simulink model "model"  (R2016a)
(part 2 of 2)

      | %<Name>
  bus13 : powerlib/Measurements/Load Flow Bus  LConnTagsString=a  Phases=single  Connectors=on one side  ID=bus13  Vbase=132000  Vref=1  Vangle=0  VLF=1  VLFb=1  VLFc=1  angleLF=0  angleLFb=0  angleLFc=0
      settings: AttributesFormatString=|
      | %<ID>
      | %<Vbase>V
      | %<VLF>pu
      | %<angleLF>deg.
      | %<Name>
  bus130 : powerlib/Measurements/Load Flow Bus  LConnTagsString=a  Phases=single  Connectors=on one side  ID=bus130  Vbase=220000  Vref=1  Vangle=0  VLF=1  VLFb=1  VLFc=1  angleLF=0  angleLFb=0  angleLFc=0
      settings: AttributesFormatString=|
      | %<ID>
      | %<Vbase>V
      | %<VLF>pu
      | %<angleLF>deg.
      | %<Name>
  bus131 : powerlib/Measurements/Load Flow Bus  LConnTagsString=a  Phases=single  Connectors=on one side  ID=bus131  Vbase=220000  Vref=1  Vangle=0  VLF=1  VLFb=1  VLFc=1  angleLF=0  angleLFb=0  angleLFc=0
      settings: AttributesFormatString=|
      | %<ID>
      | %<Vbase>V
      | %<VLF>pu
      | %<angleLF>deg.
      | %<Name>
  bus132 : powerlib/Measurements/Load Flow Bus  LConnTagsString=a  Phases=single  Connectors=on one side  ID=bus132  Vbase=220000  Vref=1  Vangle=0  VLF=1  VLFb=1  VLFc=1  angleLF=0  angleLFb=0  angleLFc=0
      settings: AttributesFormatString=|
      | %<ID>
      | %<Vbase>V
      | %<VLF>pu
      | %<angleLF>deg.
      | %<Name>
  bus133 : powerlib/Measurements/Load Flow Bus  LConnTagsString=a  Phases=single  Connectors=on one side  ID=bus133  Vbase=220000  Vref=1  Vangle=0  VLF=1  VLFb=1  VLFc=1  angleLF=0  angleLFb=0  angleLFc=0
      settings: AttributesFormatString=|
      | %<ID>
      | %<Vbase>V
      | %<VLF>pu
      | %<angleLF>deg.
      | %<Name>
  bus134 : powerlib/Measurements/Load Flow Bus  LConnTagsString=a  Phases=single  Connectors=on one side  ID=bus134  Vbase=220000  Vref=1  Vangle=0  VLF=1  VLFb=1  VLFc=1  angleLF=0  angleLFb=0  angleLFc=0
      settings: AttributesFormatString=|
      | %<ID>
      | %<Vbase>V
      | %<VLF>pu
      | %<angleLF>deg.
      | %<Name>
  bus135 : powerlib/Measurements/Load Flow Bus  LConnTagsString=a  Phases=single  Connectors=on one side  ID=bus135  Vbase=220000  Vref=1  Vangle=0  VLF=1  VLFb=1  VLFc=1  angleLF=0  angleLFb=0  angleLFc=0
      settings: AttributesFormatString=|
      | %<ID>
      | %<Vbase>V
      | %<VLF>pu
      | %<angleLF>deg.
      | %<Name>
  bus136 : powerlib/Measurements/Load Flow Bus  LConnTagsString=a  Phases=single  Connectors=on one side  ID=bus136  Vbase=220000  Vref=1  Vangle=0  VLF=1  VLFb=1  VLFc=1  angleLF=0  angleLFb=0  angleLFc=0
      settings: AttributesFormatString=|
      | %<ID>
      | %<Vbase>V
      | %<VLF>pu
      | %<angleLF>deg.
      | %<Name>
  bus137 : powerlib/Measurements/Load Flow Bus  LConnTagsString=a  Phases=single  Connectors=on one side  ID=bus137  Vbase=220000  Vref=1  Vangle=0  VLF=1  VLFb=1  VLFc=1  angleLF=0  angleLFb=0  angleLFc=0
      settings: AttributesFormatString=|
      | %<ID>
      | %<Vbase>V
      | %<VLF>pu
      | %<angleLF>deg.
      | %<Name>
  bus138 : powerlib/Measurements/Load Flow Bus  LConnTagsString=a  Phases=single  Connectors=on one side  ID=bus138  Vbase=220000  Vref=1  Vangle=0  VLF=1  VLFb=1  VLFc=1  angleLF=0  angleLFb=0  angleLFc=0
      settings: AttributesFormatString=|
      | %<ID>
      | %<Vbase>V
      | %<VLF>pu
      | %<angleLF>deg.
      | %<Name>
  bus139 : powerlib/Measurements/Load Flow Bus  LConnTagsString=a  Phases=single  Connectors=on one side  ID=bus139  Vbase=220000  Vref=1  Vangle=0  VLF=1  VLFb=1  VLFc=1  angleLF=0  angleLFb=0  angleLFc=0
      settings: AttributesFormatString=|
      | %<ID>
      | %<Vbase>V
      | %<VLF>pu
      | %<angleLF>deg.
      | %<Name>
  bus14 : powerlib/Measurements/Load Flow Bus  LConnTagsString=a  Phases=single  Connectors=on one side  ID=bus14  Vbase=132000  Vref=1  Vangle=0  VLF=1  VLFb=1  VLFc=1  angleLF=0  angleLFb=0  angleLFc=0
      settings: AttributesFormatString=|
      | %<ID>
      | %<Vbase>V
      | %<VLF>pu
      | %<angleLF>deg.
      | %<Name>
  bus140 : powerlib/Measurements/Load Flow Bus  LConnTagsString=a  Phases=single  Connectors=on one side  ID=bus140  Vbase=220000  Vref=1  Vangle=0  VLF=1  VLFb=1  VLFc=1  angleLF=0  angleLFb=0  angleLFc=0
      settings: AttributesFormatString=|
      | %<ID>
      | %<Vbase>V
      | %<VLF>pu
      | %<angleLF>deg.
      | %<Name>
  bus141 : powerlib/Measurements/Load Flow Bus  LConnTagsString=a  Phases=single  Connectors=on one side  ID=bus141  Vbase=220000  Vref=1  Vangle=0  VLF=1  VLFb=1  VLFc=1  angleLF=0  angleLFb=0  angleLFc=0
      settings: AttributesFormatString=|
      | %<ID>
      | %<Vbase>V
      | %<VLF>pu
      | %<angleLF>deg.
      | %<Name>
  bus142 : powerlib/Measurements/Load Flow Bus  LConnTagsString=a  Phases=single  Connectors=on one side  ID=bus142  Vbase=220000  Vref=1  Vangle=0  VLF=1  VLFb=1  VLFc=1  angleLF=0  angleLFb=0  angleLFc=0
      settings: AttributesFormatString=|
      | %<ID>
      | %<Vbase>V
      | %<VLF>pu
      | %<angleLF>deg.
      | %<Name>
  bus143 : powerlib/Measurements/Load Flow Bus  LConnTagsString=a  Phases=single  Connectors=on one side  ID=bus143  Vbase=220000  Vref=1  Vangle=0  VLF=1  VLFb=1  VLFc=1  angleLF=0  angleLFb=0  angleLFc=0
      settings: AttributesFormatString=|
      | %<ID>
      | %<Vbase>V
      | %<VLF>pu
      | %<angleLF>deg.
      | %<Name>
  bus144 : powerlib/Measurements/Load Flow Bus  LConnTagsString=a  Phases=single  Connectors=on one side  ID=bus144  Vbase=220000  Vref=1  Vangle=0  VLF=1  VLFb=1  VLFc=1  angleLF=0  angleLFb=0  angleLFc=0
      settings: AttributesFormatString=|
      | %<ID>
      | %<Vbase>V
      | %<VLF>pu
      | %<angleLF>deg.
      | %<Name>
  bus145 : powerlib/Measurements/Load Flow Bus  LConnTagsString=a  Phases=single  Connectors=on one side  ID=bus145  Vbase=220000  Vref=1  Vangle=0  VLF=1  VLFb=1  VLFc=1  angleLF=0  angleLFb=0  angleLFc=0
      settings: AttributesFormatString=|
      | %<ID>
      | %<Vbase>V
      | %<VLF>pu
      | %<angleLF>deg.
      | %<Name>
  bus146 : powerlib/Measurements/Load Flow Bus  LConnTagsString=a  Phases=single  Connectors=on one side  ID=bus146  Vbase=220000  Vref=1  Vangle=0  VLF=1  VLFb=1  VLFc=1  angleLF=0  angleLFb=0  angleLFc=0
      settings: AttributesFormatString=|
      | %<ID>
      | %<Vbase>V
      | %<VLF>pu
      | %<angleLF>deg.
      | %<Name>
  bus147 : powerlib/Measurements/Load Flow Bus  LConnTagsString=a  Phases=single  Connectors=on one side  ID=bus147  Vbase=220000  Vref=1  Vangle=0  VLF=1  VLFb=1  VLFc=1  angleLF=0  angleLFb=0  angleLFc=0
      settings: AttributesFormatString=|
      | %<ID>
      | %<Vbase>V
      | %<VLF>pu
      | %<angleLF>deg.
      | %<Name>
  bus148 : powerlib/Measurements/Load Flow Bus  LConnTagsString=a  Phases=single  Connectors=on one side  ID=bus148  Vbase=220000  Vref=1  Vangle=0  VLF=1  VLFb=1  VLFc=1  angleLF=0  angleLFb=0  angleLFc=0
      settings: AttributesFormatString=|
      | %<ID>
      | %<Vbase>V
      | %<VLF>pu
      | %<angleLF>deg.
      | %<Name>
  bus149 : powerlib/Measurements/Load Flow Bus  LConnTagsString=a  Phases=single  Connectors=on one side  ID=bus149  Vbase=220000  Vref=1  Vangle=0  VLF=1  VLFb=1  VLFc=1  angleLF=0  angleLFb=0  angleLFc=0
      settings: AttributesFormatString=|
      | %<ID>
      | %<Vbase>V
      | %<VLF>pu
      | %<angleLF>deg.
      | %<Name>
  bus15 : powerlib/Measurements/Load Flow Bus  LConnTagsString=a  Phases=single  Connectors=on one side  ID=bus15  Vbase=132000  Vref=1  Vangle=0  VLF=1  VLFb=1  VLFc=1  angleLF=0  angleLFb=0  angleLFc=0
      settings: AttributesFormatString=|
      | %<ID>
      | %<Vbase>V
      | %<VLF>pu
      | %<angleLF>deg.
      | %<Name>
  bus150 : powerlib/Measurements/Load Flow Bus  LConnTagsString=a  Phases=single  Connectors=on one side  ID=bus150  Vbase=220000  Vref=1  Vangle=0  VLF=1  VLFb=1  VLFc=1  angleLF=0  angleLFb=0  angleLFc=0
      settings: AttributesFormatString=|
      | %<ID>
      | %<Vbase>V
      | %<VLF>pu
      | %<angleLF>deg.
      | %<Name>
  bus151 : powerlib/Measurements/Load Flow Bus  LConnTagsString=a  Phases=single  Connectors=on one side  ID=bus151  Vbase=220000  Vref=1  Vangle=0  VLF=1  VLFb=1  VLFc=1  angleLF=0  angleLFb=0  angleLFc=0
      settings: AttributesFormatString=|
      | %<ID>
      | %<Vbase>V
      | %<VLF>pu
      | %<angleLF>deg.
      | %<Name>
  bus152 : powerlib/Measurements/Load Flow Bus  LConnTagsString=a  Phases=single  Connectors=on one side  ID=bus152  Vbase=220000  Vref=1  Vangle=0  VLF=1  VLFb=1  VLFc=1  angleLF=0  angleLFb=0  angleLFc=0
      settings: AttributesFormatString=|
      | %<ID>
      | %<Vbase>V
      | %<VLF>pu
      | %<angleLF>deg.
      | %<Name>
  bus153 : powerlib/Measurements/Load Flow Bus  LConnTagsString=a  Phases=single  Connectors=on one side  ID=bus153  Vbase=220000  Vref=1  Vangle=0  VLF=1  VLFb=1  VLFc=1  angleLF=0  angleLFb=0  angleLFc=0
      settings: AttributesFormatString=|
      | %<ID>
      | %<Vbase>V
      | %<VLF>pu
      | %<angleLF>deg.
      | %<Name>
  bus154 : powerlib/Measurements/Load Flow Bus  LConnTagsString=a  Phases=single  Connectors=on one side  ID=bus154  Vbase=220000  Vref=1  Vangle=0  VLF=1  VLFb=1  VLFc=1  angleLF=0  angleLFb=0  angleLFc=0
      settings: AttributesFormatString=|
      | %<ID>
      | %<Vbase>V
      | %<VLF>pu
      | %<angleLF>deg.
      | %<Name>
  bus155 : powerlib/Measurements/Load Flow Bus  LConnTagsString=a  Phases=single  Connectors=on one side  ID=bus155  Vbase=220000  Vref=1  Vangle=0  VLF=1  VLFb=1  VLFc=1  angleLF=0  angleLFb=0  angleLFc=0
      settings: AttributesFormatString=|
      | %<ID>
      | %<Vbase>V
      | %<VLF>pu
      | %<angleLF>deg.
      | %<Name>
  bus156 : powerlib/Measurements/Load Flow Bus  LConnTagsString=a  Phases=single  Connectors=on one side  ID=bus156  Vbase=220000  Vref=1  Vangle=0  VLF=1  VLFb=1  VLFc=1  angleLF=0  angleLFb=0  angleLFc=0
      settings: AttributesFormatString=|
      | %<ID>
      | %<Vbase>V
      | %<VLF>pu
      | %<angleLF>deg.
      | %<Name>
  bus157 : powerlib/Measurements/Load Flow Bus  LConnTagsString=a  Phases=single  Connectors=on one side  ID=bus157  Vbase=400000  Vref=1  Vangle=0  VLF=1  VLFb=1  VLFc=1  angleLF=0  angleLFb=0  angleLFc=0
      settings: AttributesFormatString=|
      | %<ID>
      | %<Vbase>V
      | %<VLF>pu
      | %<angleLF>deg.
      | %<Name>
  bus158 : powerlib/Measurements/Load Flow Bus  LConnTagsString=a  Phases=single  Connectors=on one side  ID=bus158  Vbase=400000  Vref=1  Vangle=0  VLF=1  VLFb=1  VLFc=1  angleLF=0  angleLFb=0  angleLFc=0
      settings: AttributesFormatString=|
      | %<ID>
      | %<Vbase>V
      | %<VLF>pu
      | %<angleLF>deg.
      | %<Name>
  bus159 : powerlib/Measurements/Load Flow Bus  LConnTagsString=a  Phases=single  Connectors=on one side  ID=bus159  Vbase=400000  Vref=1  Vangle=0  VLF=1  VLFb=1  VLFc=1  angleLF=0  angleLFb=0  angleLFc=0
      settings: AttributesFormatString=|
      | %<ID>
      | %<Vbase>V
      | %<VLF>pu
      | %<angleLF>deg.
      | %<Name>
  bus16 : powerlib/Measurements/Load Flow Bus  LConnTagsString=a  Phases=single  Connectors=on one side  ID=bus16  Vbase=132000  Vref=1  Vangle=0  VLF=1  VLFb=1  VLFc=1  angleLF=0  angleLFb=0  angleLFc=0
      settings: AttributesFormatString=|
      | %<ID>
      | %<Vbase>V
      | %<VLF>pu
      | %<angleLF>deg.
      | %<Name>
  bus160 : powerlib/Measurements/Load Flow Bus  LConnTagsString=a  Phases=single  Connectors=on one side  ID=bus160  Vbase=400000  Vref=1  Vangle=0  VLF=1  VLFb=1  VLFc=1  angleLF=0  angleLFb=0  angleLFc=0
      settings: AttributesFormatString=|
      | %<ID>
      | %<Vbase>V
      | %<VLF>pu
      | %<angleLF>deg.
      | %<Name>
  bus17 : powerlib/Measurements/Load Flow Bus  LConnTagsString=a  Phases=single  Connectors=on one side  ID=bus17  Vbase=132000  Vref=1  Vangle=0  VLF=1  VLFb=1  VLFc=1  angleLF=0  angleLFb=0  angleLFc=0
      settings: AttributesFormatString=|
      | %<ID>
      | %<Vbase>V
      | %<VLF>pu
      | %<angleLF>deg.
      | %<Name>
  bus18 : powerlib/Measurements/Load Flow Bus  LConnTagsString=a  Phases=single  Connectors=on one side  ID=bus18  Vbase=132000  Vref=1  Vangle=0  VLF=1  VLFb=1  VLFc=1  angleLF=0  angleLFb=0  angleLFc=0
      settings: AttributesFormatString=|
      | %<ID>
      | %<Vbase>V
      | %<VLF>pu
      | %<angleLF>deg.
      | %<Name>
  bus19 : powerlib/Measurements/Load Flow Bus  LConnTagsString=a  Phases=single  Connectors=on one side  ID=bus19  Vbase=132000  Vref=1  Vangle=0  VLF=1  VLFb=1  VLFc=1  angleLF=0  angleLFb=0  angleLFc=0
      settings: AttributesFormatString=|
      | %<ID>
      | %<Vbase>V
      | %<VLF>pu
      | %<angleLF>deg.
      | %<Name>
  bus2 : powerlib/Measurements/Load Flow Bus  LConnTagsString=a  Phases=single  Connectors=on one side  ID=bus2  Vbase=132000  Vref=1  Vangle=0  VLF=1  VLFb=1  VLFc=1  angleLF=0  angleLFb=0  angleLFc=0
      settings: AttributesFormatString=|
      | %<ID>
      | %<Vbase>V
      | %<VLF>pu
      | %<angleLF>deg.
      | %<Name>
  bus20 : powerlib/Measurements/Load Flow Bus  LConnTagsString=a  Phases=single  Connectors=on one side  ID=bus20  Vbase=132000  Vref=1  Vangle=0  VLF=1  VLFb=1  VLFc=1  angleLF=0  angleLFb=0  angleLFc=0
      settings: AttributesFormatString=|
      | %<ID>
      | %<Vbase>V
      | %<VLF>pu
      | %<angleLF>deg.
      | %<Name>
  bus21 : powerlib/Measurements/Load Flow Bus  LConnTagsString=a  Phases=single  Connectors=on one side  ID=bus21  Vbase=132000  Vref=1  Vangle=0  VLF=1  VLFb=1  VLFc=1  angleLF=0  angleLFb=0  angleLFc=0
      settings: AttributesFormatString=|
      | %<ID>
      | %<Vbase>V
      | %<VLF>pu
      | %<angleLF>deg.
      | %<Name>
  bus22 : powerlib/Measurements/Load Flow Bus  LConnTagsString=a  Phases=single  Connectors=on one side  ID=bus22  Vbase=132000  Vref=1  Vangle=0  VLF=1  VLFb=1  VLFc=1  angleLF=0  angleLFb=0  angleLFc=0
      settings: AttributesFormatString=|
      | %<ID>
      | %<Vbase>V
      | %<VLF>pu
      | %<angleLF>deg.
      | %<Name>
  bus23 : powerlib/Measurements/Load Flow Bus  LConnTagsString=a  Phases=single  Connectors=on one side  ID=bus23  Vbase=132000  Vref=1  Vangle=0  VLF=1  VLFb=1  VLFc=1  angleLF=0  angleLFb=0  angleLFc=0
      settings: AttributesFormatString=|
      | %<ID>
      | %<Vbase>V
      | %<VLF>pu
      | %<angleLF>deg.
      | %<Name>
  bus24 : powerlib/Measurements/Load Flow Bus  LConnTagsString=a  Phases=single  Connectors=on one side  ID=bus24  Vbase=132000  Vref=1  Vangle=0  VLF=1  VLFb=1  VLFc=1  angleLF=0  angleLFb=0  angleLFc=0
      settings: AttributesFormatString=|
      | %<ID>
      | %<Vbase>V
      | %<VLF>pu
      | %<angleLF>deg.
      | %<Name>
  bus25 : powerlib/Measurements/Load Flow Bus  LConnTagsString=a  Phases=single  Connectors=on one side  ID=bus25  Vbase=132000  Vref=1  Vangle=0  VLF=1  VLFb=1  VLFc=1  angleLF=0  angleLFb=0  angleLFc=0
      settings: AttributesFormatString=|
      | %<ID>
      | %<Vbase>V
      | %<VLF>pu
      | %<angleLF>deg.
      | %<Name>
  bus26 : powerlib/Measurements/Load Flow Bus  LConnTagsString=a  Phases=single  Connectors=on one side  ID=bus26  Vbase=220000  Vref=1  Vangle=0  VLF=1  VLFb=1  VLFc=1  angleLF=0  angleLFb=0  angleLFc=0
      settings: AttributesFormatString=|
      | %<ID>
      | %<Vbase>V
      | %<VLF>pu
      | %<angleLF>deg.
      | %<Name>
  bus27 : powerlib/Measurements/Load Flow Bus  LConnTagsString=a  Phases=single  Connectors=on one side  ID=bus27  Vbase=220000  Vref=1  Vangle=0  VLF=1  VLFb=1  VLFc=1  angleLF=0  angleLFb=0  angleLFc=0
      settings: AttributesFormatString=|
      | %<ID>
      | %<Vbase>V
      | %<VLF>pu
      | %<angleLF>deg.
      | %<Name>
  bus28 : powerlib/Measurements/Load Flow Bus  LConnTagsString=a  Phases=single  Connectors=on one side  ID=bus28  Vbase=220000  Vref=1  Vangle=0  VLF=1  VLFb=1  VLFc=1  angleLF=0  angleLFb=0  angleLFc=0
      settings: AttributesFormatString=|
      | %<ID>
      | %<Vbase>V
      | %<VLF>pu
      | %<angleLF>deg.
      | %<Name>
  bus29 : powerlib/Measurements/Load Flow Bus  LConnTagsString=a  Phases=single  Connectors=on one side  ID=bus29  Vbase=220000  Vref=1  Vangle=0  VLF=1  VLFb=1  VLFc=1  angleLF=0  angleLFb=0  angleLFc=0
      settings: AttributesFormatString=|
      | %<ID>
      | %<Vbase>V
      | %<VLF>pu
      | %<angleLF>deg.
      | %<Name>
  bus3 : powerlib/Measurements/Load Flow Bus  LConnTagsString=a  Phases=single  Connectors=on one side  ID=bus3  Vbase=132000  Vref=1  Vangle=0  VLF=1  VLFb=1  VLFc=1  angleLF=0  angleLFb=0  angleLFc=0
      settings: AttributesFormatString=|
      | %<ID>
      | %<Vbase>V
      | %<VLF>pu
      | %<angleLF>deg.
      | %<Name>
  bus30 : powerlib/Measurements/Load Flow Bus  LConnTagsString=a  Phases=single  Connectors=on one side  ID=bus30  Vbase=220000  Vref=1  Vangle=0  VLF=1  VLFb=1  VLFc=1  angleLF=0  angleLFb=0  angleLFc=0
      settings: AttributesFormatString=|
      | %<ID>
      | %<Vbase>V
      | %<VLF>pu
      | %<angleLF>deg.
      | %<Name>
  bus31 : powerlib/Measurements/Load Flow Bus  LConnTagsString=a  Phases=single  Connectors=on one side  ID=bus31  Vbase=220000  Vref=1  Vangle=0  VLF=1  VLFb=1  VLFc=1  angleLF=0  angleLFb=0  angleLFc=0
      settings: AttributesFormatString=|
      | %<ID>
      | %<Vbase>V
      | %<VLF>pu
      | %<angleLF>deg.
      | %<Name>
  bus32 : powerlib/Measurements/Load Flow Bus  LConnTagsString=a  Phases=single  Connectors=on one side  ID=bus32  Vbase=220000  Vref=1  Vangle=0  VLF=1  VLFb=1  VLFc=1  angleLF=0  angleLFb=0  angleLFc=0
      settings: AttributesFormatString=|
      | %<ID>
      | %<Vbase>V
      | %<VLF>pu
      | %<angleLF>deg.
      | %<Name>
  bus33 : powerlib/Measurements/Load Flow Bus  LConnTagsString=a  Phases=single  Connectors=on one side  ID=bus33  Vbase=220000  Vref=1  Vangle=0  VLF=1  VLFb=1  VLFc=1  angleLF=0  angleLFb=0  angleLFc=0
      settings: AttributesFormatString=|
      | %<ID>
      | %<Vbase>V
      | %<VLF>pu
      | %<angleLF>deg.
      | %<Name>
  bus34 : powerlib/Measurements/Load Flow Bus  LConnTagsString=a  Phases=single  Connectors=on one side  ID=bus34  Vbase=220000  Vref=1  Vangle=0  VLF=1  VLFb=1  VLFc=1  angleLF=0  angleLFb=0  angleLFc=0
      settings: AttributesFormatString=|
      | %<ID>
      | %<Vbase>V
      | %<VLF>pu
      | %<angleLF>deg.
      | %<Name>
  bus35 : powerlib/Measurements/Load Flow Bus  LConnTagsString=a  Phases=single  Connectors=on one side  ID=bus35  Vbase=220000  Vref=1  Vangle=0  VLF=1  VLFb=1  VLFc=1  angleLF=0  angleLFb=0  angleLFc=0
      settings: AttributesFormatString=|
      | %<ID>
      | %<Vbase>V
      | %<VLF>pu
      | %<angleLF>deg.
      | %<Name>
  bus36 : powerlib/Measurements/Load Flow Bus  LConnTagsString=a  Phases=single  Connectors=on one side  ID=bus36  Vbase=220000  Vref=1  Vangle=0  VLF=1  VLFb=1  VLFc=1  angleLF=0  angleLFb=0  angleLFc=0
      settings: AttributesFormatString=|
      | %<ID>
      | %<Vbase>V
      | %<VLF>pu
      | %<angleLF>deg.
      | %<Name>
  bus37 : powerlib/Measurements/Load Flow Bus  LConnTagsString=a  Phases=single  Connectors=on one side  ID=bus37  Vbase=220000  Vref=1  Vangle=0  VLF=1  VLFb=1  VLFc=1  angleLF=0  angleLFb=0  angleLFc=0
      settings: AttributesFormatString=|
      | %<ID>
      | %<Vbase>V
      | %<VLF>pu
      | %<angleLF>deg.
      | %<Name>
  bus38 : powerlib/Measurements/Load Flow Bus  LConnTagsString=a  Phases=single  Connectors=on one side  ID=bus38  Vbase=220000  Vref=1  Vangle=0  VLF=1  VLFb=1  VLFc=1  angleLF=0  angleLFb=0  angleLFc=0
      settings: AttributesFormatString=|
      | %<ID>
      | %<Vbase>V
      | %<VLF>pu
      | %<angleLF>deg.
      | %<Name>
  bus39 : powerlib/Measurements/Load Flow Bus  LConnTagsString=a  Phases=single  Connectors=on one side  ID=bus39  Vbase=220000  Vref=1  Vangle=0  VLF=1  VLFb=1  VLFc=1  angleLF=0  angleLFb=0  angleLFc=0
      settings: AttributesFormatString=|
      | %<ID>
      | %<Vbase>V
      | %<VLF>pu
      | %<angleLF>deg.
      | %<Name>
  bus4 : powerlib/Measurements/Load Flow Bus  LConnTagsString=a  Phases=single  Connectors=on one side  ID=bus4  Vbase=132000  Vref=1  Vangle=0  VLF=1  VLFb=1  VLFc=1  angleLF=0  angleLFb=0  angleLFc=0
      settings: AttributesFormatString=|
      | %<ID>
      | %<Vbase>V
      | %<VLF>pu
      | %<angleLF>deg.
      | %<Name>
  bus40 : powerlib/Measurements/Load Flow Bus  LConnTagsString=a  Phases=single  Connectors=on one side  ID=bus40  Vbase=220000  Vref=1  Vangle=0  VLF=1  VLFb=1  VLFc=1  angleLF=0  angleLFb=0  angleLFc=0
      settings: AttributesFormatString=|
      | %<ID>
      | %<Vbase>V
      | %<VLF>pu
      | %<angleLF>deg.
      | %<Name>
  bus41 : powerlib/Measurements/Load Flow Bus  LConnTagsString=a  Phases=single  Connectors=on one side  ID=bus41  Vbase=220000  Vref=1  Vangle=0  VLF=1  VLFb=1  VLFc=1  angleLF=0  angleLFb=0  angleLFc=0
      settings: AttributesFormatString=|
      | %<ID>
      | %<Vbase>V
      | %<VLF>pu
      | %<angleLF>deg.
      | %<Name>
  bus42 : powerlib/Measurements/Load Flow Bus  LConnTagsString=a  Phases=single  Connectors=on one side  ID=bus42  Vbase=220000  Vref=1  Vangle=0  VLF=1  VLFb=1  VLFc=1  angleLF=0  angleLFb=0  angleLFc=0
      settings: AttributesFormatString=|
      | %<ID>
      | %<Vbase>V
      | %<VLF>pu
      | %<angleLF>deg.
      | %<Name>
  bus43 : powerlib/Measurements/Load Flow Bus  LConnTagsString=a  Phases=single  Connectors=on one side  ID=bus43  Vbase=220000  Vref=1  Vangle=0  VLF=1  VLFb=1  VLFc=1  angleLF=0  angleLFb=0  angleLFc=0
      settings: AttributesFormatString=|
      | %<ID>
      | %<Vbase>V
      | %<VLF>pu
      | %<angleLF>deg.
      | %<Name>
  bus44 : powerlib/Measurements/Load Flow Bus  LConnTagsString=a  Phases=single  Connectors=on one side  ID=bus44  Vbase=220000  Vref=1  Vangle=0  VLF=1  VLFb=1  VLFc=1  angleLF=0  angleLFb=0  angleLFc=0
      settings: AttributesFormatString=|
      | %<ID>
      | %<Vbase>V
      | %<VLF>pu
      | %<angleLF>deg.
      | %<Name>
  bus45 : powerlib/Measurements/Load Flow Bus  LConnTagsString=a  Phases=single  Connectors=on one side  ID=bus45  Vbase=220000  Vref=1  Vangle=0  VLF=1  VLFb=1  VLFc=1  angleLF=0  angleLFb=0  angleLFc=0
      settings: AttributesFormatString=|
      | %<ID>
      | %<Vbase>V
      | %<VLF>pu
      | %<angleLF>deg.
      | %<Name>
  bus46 : powerlib/Measurements/Load Flow Bus  LConnTagsString=a  Phases=single  Connectors=on one side  ID=bus46  Vbase=220000  Vref=1  Vangle=0  VLF=1  VLFb=1  VLFc=1  angleLF=0  angleLFb=0  angleLFc=0
      settings: AttributesFormatString=|
      | %<ID>
      | %<Vbase>V
      | %<VLF>pu
      | %<angleLF>deg.
      | %<Name>
  bus47 : powerlib/Measurements/Load Flow Bus  LConnTagsString=a  Phases=single  Connectors=on one side  ID=bus47  Vbase=220000  Vref=1  Vangle=0  VLF=1  VLFb=1  VLFc=1  angleLF=0  angleLFb=0  angleLFc=0
      settings: AttributesFormatString=|
      | %<ID>
      | %<Vbase>V
      | %<VLF>pu
      | %<angleLF>deg.
      | %<Name>
  bus48 : powerlib/Measurements/Load Flow Bus  LConnTagsString=a  Phases=single  Connectors=on one side  ID=bus48  Vbase=220000  Vref=1  Vangle=0  VLF=1  VLFb=1  VLFc=1  angleLF=0  angleLFb=0  angleLFc=0
      settings: AttributesFormatString=|
      | %<ID>
      | %<Vbase>V
      | %<VLF>pu
      | %<angleLF>deg.
      | %<Name>
  bus49 : powerlib/Measurements/Load Flow Bus  LConnTagsString=a  Phases=single  Connectors=on one side  ID=bus49  Vbase=220000  Vref=1  Vangle=0  VLF=1  VLFb=1  VLFc=1  angleLF=0  angleLFb=0  angleLFc=0
      settings: AttributesFormatString=|
      | %<ID>
      | %<Vbase>V
      | %<VLF>pu
      | %<angleLF>deg.
      | %<Name>
  bus5 : powerlib/Measurements/Load Flow Bus  LConnTagsString=a  Phases=single  Connectors=on one side  ID=bus5  Vbase=132000  Vref=1  Vangle=0  VLF=1  VLFb=1  VLFc=1  angleLF=0  angleLFb=0  angleLFc=0
      settings: AttributesFormatString=|
      | %<ID>
      | %<Vbase>V
      | %<VLF>pu
      | %<angleLF>deg.
      | %<Name>
  bus50 : powerlib/Measurements/Load Flow Bus  LConnTagsString=a  Phases=single  Connectors=on one side  ID=bus50  Vbase=220000  Vref=1  Vangle=0  VLF=1  VLFb=1  VLFc=1  angleLF=0  angleLFb=0  angleLFc=0
      settings: AttributesFormatString=|
      | %<ID>
      | %<Vbase>V
      | %<VLF>pu
      | %<angleLF>deg.
      | %<Name>
  bus51 : powerlib/Measurements/Load Flow Bus  LConnTagsString=a  Phases=single  Connectors=on one side  ID=bus51  Vbase=220000  Vref=1  Vangle=0  VLF=1  VLFb=1  VLFc=1  angleLF=0  angleLFb=0  angleLFc=0
      settings: AttributesFormatString=|
      | %<ID>
      | %<Vbase>V
      | %<VLF>pu
      | %<angleLF>deg.
      | %<Name>
  bus52 : powerlib/Measurements/Load Flow Bus  LConnTagsString=a  Phases=single  Connectors=on one side  ID=bus52  Vbase=220000  Vref=1  Vangle=0  VLF=1  VLFb=1  VLFc=1  angleLF=0  angleLFb=0  angleLFc=0
      settings: AttributesFormatString=|
      | %<ID>
      | %<Vbase>V
      | %<VLF>pu
      | %<angleLF>deg.
      | %<Name>
  bus53 : powerlib/Measurements/Load Flow Bus  LConnTagsString=a  Phases=single  Connectors=on one side  ID=bus53  Vbase=220000  Vref=1  Vangle=0  VLF=1  VLFb=1  VLFc=1  angleLF=0  angleLFb=0  angleLFc=0
      settings: AttributesFormatString=|
      | %<ID>
      | %<Vbase>V
      | %<VLF>pu
      | %<angleLF>deg.
      | %<Name>
  bus54 : powerlib/Measurements/Load Flow Bus  LConnTagsString=a  Phases=single  Connectors=on one side  ID=bus54  Vbase=220000  Vref=1  Vangle=0  VLF=1  VLFb=1  VLFc=1  angleLF=0  angleLFb=0  angleLFc=0
      settings: AttributesFormatString=|
      | %<ID>
      | %<Vbase>V
      | %<VLF>pu
      | %<angleLF>deg.
      | %<Name>
  bus55 : powerlib/Measurements/Load Flow Bus  LConnTagsString=a  Phases=single  Connectors=on one side  ID=bus55  Vbase=220000  Vref=1  Vangle=0  VLF=1  VLFb=1  VLFc=1  angleLF=0  angleLFb=0  angleLFc=0
      settings: AttributesFormatString=|
      | %<ID>
      | %<Vbase>V
      | %<VLF>pu
      | %<angleLF>deg.
      | %<Name>
  bus56 : powerlib/Measurements/Load Flow Bus  LConnTagsString=a  Phases=single  Connectors=on one side  ID=bus56  Vbase=220000  Vref=1  Vangle=0  VLF=1  VLFb=1  VLFc=1  angleLF=0  angleLFb=0  angleLFc=0
      settings: AttributesFormatString=|
      | %<ID>
      | %<Vbase>V
      | %<VLF>pu
      | %<angleLF>deg.
      | %<Name>
  bus57 : powerlib/Measurements/Load Flow Bus  LConnTagsString=a  Phases=single  Connectors=on one side  ID=bus57  Vbase=220000  Vref=1  Vangle=0  VLF=1  VLFb=1  VLFc=1  angleLF=0  angleLFb=0  angleLFc=0
      settings: AttributesFormatString=|
      | %<ID>
      | %<Vbase>V
      | %<VLF>pu
      | %<angleLF>deg.
      | %<Name>
  bus58 : powerlib/Measurements/Load Flow Bus  LConnTagsString=a  Phases=single  Connectors=on one side  ID=bus58  Vbase=220000  Vref=1  Vangle=0  VLF=1  VLFb=1  VLFc=1  angleLF=0  angleLFb=0  angleLFc=0
      settings: AttributesFormatString=|
      | %<ID>
      | %<Vbase>V
      | %<VLF>pu
      | %<angleLF>deg.
      | %<Name>
  bus59 : powerlib/Measurements/Load Flow Bus  LConnTagsString=a  Phases=single  Connectors=on one side  ID=bus59  Vbase=220000  Vref=1  Vangle=0  VLF=1  VLFb=1  VLFc=1  angleLF=0  angleLFb=0  angleLFc=0
      settings: AttributesFormatString=|
      | %<ID>
      | %<Vbase>V
      | %<VLF>pu
      | %<angleLF>deg.
      | %<Name>
  bus6 : powerlib/Measurements/Load Flow Bus  LConnTagsString=a  Phases=single  Connectors=on one side  ID=bus6  Vbase=132000  Vref=1  Vangle=0  VLF=1  VLFb=1  VLFc=1  angleLF=0  angleLFb=0  angleLFc=0
      settings: AttributesFormatString=|
      | %<ID>
      | %<Vbase>V
      | %<VLF>pu
      | %<angleLF>deg.
      | %<Name>
  bus60 : powerlib/Measurements/Load Flow Bus  LConnTagsString=a  Phases=single  Connectors=on one side  ID=bus60  Vbase=220000  Vref=1  Vangle=0  VLF=1  VLFb=1  VLFc=1  angleLF=0  angleLFb=0  angleLFc=0
      settings: AttributesFormatString=|
      | %<ID>
      | %<Vbase>V
      | %<VLF>pu
      | %<angleLF>deg.
      | %<Name>
  bus61 : powerlib/Measurements/Load Flow Bus  LConnTagsString=a  Phases=single  Connectors=on one side  ID=bus61  Vbase=220000  Vref=1  Vangle=0  VLF=1  VLFb=1  VLFc=1  angleLF=0  angleLFb=0  angleLFc=0
      settings: AttributesFormatString=|
      | %<ID>
      | %<Vbase>V
      | %<VLF>pu
      | %<angleLF>deg.
      | %<Name>
  bus62 : powerlib/Measurements/Load Flow Bus  LConnTagsString=a  Phases=single  Connectors=on one side  ID=bus62  Vbase=220000  Vref=1  Vangle=0  VLF=1  VLFb=1  VLFc=1  angleLF=0  angleLFb=0  angleLFc=0
      settings: AttributesFormatString=|
      | %<ID>
      | %<Vbase>V
      | %<VLF>pu
      | %<angleLF>deg.
      | %<Name>
  bus63 : powerlib/Measurements/Load Flow Bus  LConnTagsString=a  Phases=single  Connectors=on one side  ID=bus63  Vbase=220000  Vref=1  Vangle=0  VLF=1  VLFb=1  VLFc=1  angleLF=0  angleLFb=0  angleLFc=0
      settings: AttributesFormatString=|
      | %<ID>
      | %<Vbase>V
      | %<VLF>pu
      | %<angleLF>deg.
      | %<Name>
  bus64 : powerlib/Measurements/Load Flow Bus  LConnTagsString=a  Phases=single  Connectors=on one side  ID=bus64  Vbase=220000  Vref=1  Vangle=0  VLF=1  VLFb=1  VLFc=1  angleLF=0  angleLFb=0  angleLFc=0
      settings: AttributesFormatString=|
      | %<ID>
      | %<Vbase>V
      | %<VLF>pu
      | %<angleLF>deg.
      | %<Name>
  bus65 : powerlib/Measurements/Load Flow Bus  LConnTagsString=a  Phases=single  Connectors=on one side  ID=bus65  Vbase=220000  Vref=1  Vangle=0  VLF=1  VLFb=1  VLFc=1  angleLF=0  angleLFb=0  angleLFc=0
      settings: AttributesFormatString=|
      | %<ID>
      | %<Vbase>V
      | %<VLF>pu
      | %<angleLF>deg.
      | %<Name>
  bus66 : powerlib/Measurements/Load Flow Bus  LConnTagsString=a  Phases=single  Connectors=on one side  ID=bus66  Vbase=220000  Vref=1  Vangle=0  VLF=1  VLFb=1  VLFc=1  angleLF=0  angleLFb=0  angleLFc=0
      settings: AttributesFormatString=|
      | %<ID>
      | %<Vbase>V
      | %<VLF>pu
      | %<angleLF>deg.
      | %<Name>
  bus67 : powerlib/Measurements/Load Flow Bus  LConnTagsString=a  Phases=single  Connectors=on one side  ID=bus67  Vbase=220000  Vref=1  Vangle=0  VLF=1  VLFb=1  VLFc=1  angleLF=0  angleLFb=0  angleLFc=0
      settings: AttributesFormatString=|
      | %<ID>
      | %<Vbase>V
      | %<VLF>pu
      | %<angleLF>deg.
      | %<Name>
  bus68 : powerlib/Measurements/Load Flow Bus  LConnTagsString=a  Phases=single  Connectors=on one side  ID=bus68  Vbase=220000  Vref=1  Vangle=0  VLF=1  VLFb=1  VLFc=1  angleLF=0  angleLFb=0  angleLFc=0
      settings: AttributesFormatString=|
      | %<ID>
      | %<Vbase>V
      | %<VLF>pu
      | %<angleLF>deg.
      | %<Name>
  bus69 : powerlib/Measurements/Load Flow Bus  LConnTagsString=a  Phases=single  Connectors=on one side  ID=bus69  Vbase=220000  Vref=1  Vangle=0  VLF=1  VLFb=1  VLFc=1  angleLF=0  angleLFb=0  angleLFc=0
      settings: AttributesFormatString=|
      | %<ID>
      | %<Vbase>V
      | %<VLF>pu
      | %<angleLF>deg.
      | %<Name>
  bus7 : powerlib/Measurements/Load Flow Bus  LConnTagsString=a  Phases=single  Connectors=on one side  ID=bus7  Vbase=132000  Vref=1  Vangle=0  VLF=1  VLFb=1  VLFc=1  angleLF=0  angleLFb=0  angleLFc=0
      settings: AttributesFormatString=|
      | %<ID>
      | %<Vbase>V
      | %<VLF>pu
      | %<angleLF>deg.
      | %<Name>
  bus70 : powerlib/Measurements/Load Flow Bus  LConnTagsString=a  Phases=single  Connectors=on one side  ID=bus70  Vbase=220000  Vref=1  Vangle=0  VLF=1  VLFb=1  VLFc=1  angleLF=0  angleLFb=0  angleLFc=0
      settings: AttributesFormatString=|
      | %<ID>
      | %<Vbase>V
      | %<VLF>pu
      | %<angleLF>deg.
      | %<Name>
  bus71 : powerlib/Measurements/Load Flow Bus  LConnTagsString=a  Phases=single  Connectors=on one side  ID=bus71  Vbase=220000  Vref=1  Vangle=0  VLF=1  VLFb=1  VLFc=1  angleLF=0  angleLFb=0  angleLFc=0
      settings: AttributesFormatString=|
      | %<ID>
      | %<Vbase>V
      | %<VLF>pu
      | %<angleLF>deg.
      | %<Name>
  bus72 : powerlib/Measurements/Load Flow Bus  LConnTagsString=a  Phases=single  Connectors=on one side  ID=bus72  Vbase=220000  Vref=1  Vangle=0  VLF=1  VLFb=1  VLFc=1  angleLF=0  angleLFb=0  angleLFc=0
      settings: AttributesFormatString=|
      | %<ID>
      | %<Vbase>V
      | %<VLF>pu
      | %<angleLF>deg.
      | %<Name>
  bus73 : powerlib/Measurements/Load Flow Bus  LConnTagsString=a  Phases=single  Connectors=on one side  ID=bus73  Vbase=220000  Vref=1  Vangle=0  VLF=1  VLFb=1  VLFc=1  angleLF=0  angleLFb=0  angleLFc=0
      settings: AttributesFormatString=|
      | %<ID>
      | %<Vbase>V
      | %<VLF>pu
      | %<angleLF>deg.
      | %<Name>
  bus74 : powerlib/Measurements/Load Flow Bus  LConnTagsString=a  Phases=single  Connectors=on one side  ID=bus74  Vbase=220000  Vref=1  Vangle=0  VLF=1  VLFb=1  VLFc=1  angleLF=0  angleLFb=0  angleLFc=0
      settings: AttributesFormatString=|
      | %<ID>
      | %<Vbase>V
      | %<VLF>pu
      | %<angleLF>deg.
      | %<Name>
  bus75 : powerlib/Measurements/Load Flow Bus  LConnTagsString=a  Phases=single  Connectors=on one side  ID=bus75  Vbase=220000  Vref=1  Vangle=0  VLF=1  VLFb=1  VLFc=1  angleLF=0  angleLFb=0  angleLFc=0
      settings: AttributesFormatString=|
      | %<ID>
      | %<Vbase>V
      | %<VLF>pu
      | %<angleLF>deg.
      | %<Name>
  bus76 : powerlib/Measurements/Load Flow Bus  LConnTagsString=a  Phases=single  Connectors=on one side  ID=bus76  Vbase=220000  Vref=1  Vangle=0  VLF=1  VLFb=1  VLFc=1  angleLF=0  angleLFb=0  angleLFc=0
      settings: AttributesFormatString=|
      | %<ID>
      | %<Vbase>V
      | %<VLF>pu
      | %<angleLF>deg.
      | %<Name>
  bus77 : powerlib/Measurements/Load Flow Bus  LConnTagsString=a  Phases=single  Connectors=on one side  ID=bus77  Vbase=220000  Vref=1  Vangle=0  VLF=1  VLFb=1  VLFc=1  angleLF=0  angleLFb=0  angleLFc=0
      settings: AttributesFormatString=|
      | %<ID>
      | %<Vbase>V
      | %<VLF>pu
      | %<angleLF>deg.
      | %<Name>
  bus78 : powerlib/Measurements/Load Flow Bus  LConnTagsString=a  Phases=single  Connectors=on one side  ID=bus78  Vbase=220000  Vref=1  Vangle=0  VLF=1  VLFb=1  VLFc=1  angleLF=0  angleLFb=0  angleLFc=0
      settings: AttributesFormatString=|
      | %<ID>
      | %<Vbase>V
      | %<VLF>pu
      | %<angleLF>deg.
      | %<Name>
  bus79 : powerlib/Measurements/Load Flow Bus  LConnTagsString=a  Phases=single  Connectors=on one side  ID=bus79  Vbase=220000  Vref=1  Vangle=0  VLF=1  VLFb=1  VLFc=1  angleLF=0  angleLFb=0  angleLFc=0
      settings: AttributesFormatString=|
      | %<ID>
      | %<Vbase>V
      | %<VLF>pu
      | %<angleLF>deg.
      | %<Name>
  bus8 : powerlib/Measurements/Load Flow Bus  LConnTagsString=a  Phases=single  Connectors=on one side  ID=bus8  Vbase=132000  Vref=1  Vangle=0  VLF=1  VLFb=1  VLFc=1  angleLF=0  angleLFb=0  angleLFc=0
      settings: AttributesFormatString=|
      | %<ID>
      | %<Vbase>V
      | %<VLF>pu
      | %<angleLF>deg.
      | %<Name>
  bus80 : powerlib/Measurements/Load Flow Bus  LConnTagsString=a  Phases=single  Connectors=on one side  ID=bus80  Vbase=220000  Vref=1  Vangle=0  VLF=1  VLFb=1  VLFc=1  angleLF=0  angleLFb=0  angleLFc=0
      settings: AttributesFormatString=|
      | %<ID>
      | %<Vbase>V
      | %<VLF>pu
      | %<angleLF>deg.
      | %<Name>
  bus81 : powerlib/Measurements/Load Flow Bus  LConnTagsString=a  Phases=single  Connectors=on one side  ID=bus81  Vbase=220000  Vref=1  Vangle=0  VLF=1  VLFb=1  VLFc=1  angleLF=0  angleLFb=0  angleLFc=0
      settings: AttributesFormatString=|
      | %<ID>
      | %<Vbase>V
      | %<VLF>pu
      | %<angleLF>deg.
      | %<Name>
  bus82 : powerlib/Measurements/Load Flow Bus  LConnTagsString=a  Phases=single  Connectors=on one side  ID=bus82  Vbase=400000  Vref=1  Vangle=0  VLF=1  VLFb=1  VLFc=1  angleLF=0  angleLFb=0  angleLFc=0
      settings: AttributesFormatString=|
      | %<ID>
      | %<Vbase>V
      | %<VLF>pu
      | %<angleLF>deg.
      | %<Name>
  bus83 : powerlib/Measurements/Load Flow Bus  LConnTagsString=a  Phases=single  Connectors=on one side  ID=bus83  Vbase=400000  Vref=1  Vangle=0  VLF=1  VLFb=1  VLFc=1  angleLF=0  angleLFb=0  angleLFc=0
      settings: AttributesFormatString=|
      | %<ID>
      | %<Vbase>V
      | %<VLF>pu
      | %<angleLF>deg.
      | %<Name>
  bus84 : powerlib/Measurements/Load Flow Bus  LConnTagsString=a  Phases=single  Connectors=on one side  ID=bus84  Vbase=400000  Vref=1  Vangle=0  VLF=1  VLFb=1  VLFc=1  angleLF=0  angleLFb=0  angleLFc=0
      settings: AttributesFormatString=|
      | %<ID>
      | %<Vbase>V
      | %<VLF>pu
      | %<angleLF>deg.
      | %<Name>
  bus85 : powerlib/Measurements/Load Flow Bus  LConnTagsString=a  Phases=single  Connectors=on one side  ID=bus85  Vbase=400000  Vref=1  Vangle=0  VLF=1  VLFb=1  VLFc=1  angleLF=0  angleLFb=0  angleLFc=0
      settings: AttributesFormatString=|
      | %<ID>
      | %<Vbase>V
      | %<VLF>pu
      | %<angleLF>deg.
      | %<Name>
  bus86 : powerlib/Measurements/Load Flow Bus  LConnTagsString=a  Phases=single  Connectors=on one side  ID=bus86  Vbase=400000  Vref=1  Vangle=0  VLF=1  VLFb=1  VLFc=1  angleLF=0  angleLFb=0  angleLFc=0
      settings: AttributesFormatString=|
      | %<ID>
      | %<Vbase>V
      | %<VLF>pu
      | %<angleLF>deg.
      | %<Name>
  bus87 : powerlib/Measurements/Load Flow Bus  LConnTagsString=a  Phases=single  Connectors=on one side  ID=bus87  Vbase=400000  Vref=1  Vangle=0  VLF=1  VLFb=1  VLFc=1  angleLF=0  angleLFb=0  angleLFc=0
      settings: AttributesFormatString=|
      | %<ID>
      | %<Vbase>V
      | %<VLF>pu
      | %<angleLF>deg.
      | %<Name>
  bus88 : powerlib/Measurements/Load Flow Bus  LConnTagsString=a  Phases=single  Connectors=on one side  ID=bus88  Vbase=400000  Vref=1  Vangle=0  VLF=1  VLFb=1  VLFc=1  angleLF=0  angleLFb=0  angleLFc=0
      settings: AttributesFormatString=|
      | %<ID>
      | %<Vbase>V
      | %<VLF>pu
      | %<angleLF>deg.
      | %<Name>
  bus89 : powerlib/Measurements/Load Flow Bus  LConnTagsString=a  Phases=single  Connectors=on one side  ID=bus89  Vbase=132000  Vref=1  Vangle=0  VLF=1  VLFb=1  VLFc=1  angleLF=0  angleLFb=0  angleLFc=0
      settings: AttributesFormatString=|
      | %<ID>
      | %<Vbase>V
      | %<VLF>pu
      | %<angleLF>deg.
      | %<Name>
  bus9 : powerlib/Measurements/Load Flow Bus  LConnTagsString=a  Phases=single  Connectors=on one side  ID=bus9  Vbase=132000  Vref=1  Vangle=0  VLF=1  VLFb=1  VLFc=1  angleLF=0  angleLFb=0  angleLFc=0
      settings: AttributesFormatString=|
      | %<ID>
      | %<Vbase>V
      | %<VLF>pu
      | %<angleLF>deg.
      | %<Name>
  bus90 : powerlib/Measurements/Load Flow Bus  LConnTagsString=a  Phases=single  Connectors=on one side  ID=bus90  Vbase=132000  Vref=1  Vangle=0  VLF=1  VLFb=1  VLFc=1  angleLF=0  angleLFb=0  angleLFc=0
      settings: AttributesFormatString=|
      | %<ID>
      | %<Vbase>V
      | %<VLF>pu
      | %<angleLF>deg.
      | %<Name>
  bus91 : powerlib/Measurements/Load Flow Bus  LConnTagsString=a  Phases=single  Connectors=on one side  ID=bus91  Vbase=132000  Vref=1  Vangle=0  VLF=1  VLFb=1  VLFc=1  angleLF=0  angleLFb=0  angleLFc=0
      settings: AttributesFormatString=|
      | %<ID>
      | %<Vbase>V
      | %<VLF>pu
      | %<angleLF>deg.
      | %<Name>
  bus92 : powerlib/Measurements/Load Flow Bus  LConnTagsString=a  Phases=single  Connectors=on one side  ID=bus92  Vbase=132000  Vref=1  Vangle=0  VLF=1  VLFb=1  VLFc=1  angleLF=0  angleLFb=0  angleLFc=0
      settings: AttributesFormatString=|
      | %<ID>
      | %<Vbase>V
      | %<VLF>pu
      | %<angleLF>deg.
      | %<Name>
  bus93 : powerlib/Measurements/Load Flow Bus  LConnTagsString=a  Phases=single  Connectors=on one side  ID=bus93  Vbase=132000  Vref=1  Vangle=0  VLF=1  VLFb=1  VLFc=1  angleLF=0  angleLFb=0  angleLFc=0
      settings: AttributesFormatString=|
      | %<ID>
      | %<Vbase>V
      | %<VLF>pu
      | %<angleLF>deg.
      | %<Name>
  bus94 : powerlib/Measurements/Load Flow Bus  LConnTagsString=a  Phases=single  Connectors=on one side  ID=bus94  Vbase=132000  Vref=1  Vangle=0  VLF=1  VLFb=1  VLFc=1  angleLF=0  angleLFb=0  angleLFc=0
      settings: AttributesFormatString=|
      | %<ID>
      | %<Vbase>V
      | %<VLF>pu
      | %<angleLF>deg.
      | %<Name>
  bus95 : powerlib/Measurements/Load Flow Bus  LConnTagsString=a  Phases=single  Connectors=on one side  ID=bus95  Vbase=132000  Vref=1  Vangle=0  VLF=1  VLFb=1  VLFc=1  angleLF=0  angleLFb=0  angleLFc=0
      settings: AttributesFormatString=|
      | %<ID>
      | %<Vbase>V
      | %<VLF>pu
      | %<angleLF>deg.
      | %<Name>
  bus96 : powerlib/Measurements/Load Flow Bus  LConnTagsString=a  Phases=single  Connectors=on one side  ID=bus96  Vbase=132000  Vref=1  Vangle=0  VLF=1  VLFb=1  VLFc=1  angleLF=0  angleLFb=0  angleLFc=0
      settings: AttributesFormatString=|
      | %<ID>
      | %<Vbase>V
      | %<VLF>pu
      | %<angleLF>deg.
      | %<Name>
  bus97 : powerlib/Measurements/Load Flow Bus  LConnTagsString=a  Phases=single  Connectors=on one side  ID=bus97  Vbase=132000  Vref=1  Vangle=0  VLF=1  VLFb=1  VLFc=1  angleLF=0  angleLFb=0  angleLFc=0
      settings: AttributesFormatString=|
      | %<ID>
      | %<Vbase>V
      | %<VLF>pu
      | %<angleLF>deg.
      | %<Name>
  bus98 : powerlib/Measurements/Load Flow Bus  LConnTagsString=a  Phases=single  Connectors=on one side  ID=bus98  Vbase=132000  Vref=1  Vangle=0  VLF=1  VLFb=1  VLFc=1  angleLF=0  angleLFb=0  angleLFc=0
      settings: AttributesFormatString=|
      | %<ID>
      | %<Vbase>V
      | %<VLF>pu
      | %<angleLF>deg.
      | %<Name>
  bus99 : powerlib/Measurements/Load Flow Bus  LConnTagsString=a  Phases=single  Connectors=on one side  ID=bus99  Vbase=132000  Vref=1  Vangle=0  VLF=1  VLFb=1  VLFc=1  angleLF=0  angleLFb=0  angleLFc=0
      settings: AttributesFormatString=|
      | %<ID>
      | %<Vbase>V
      | %<VLF>pu
      | %<angleLF>deg.
      | %<Name>
  powergui : powerlib/powergui  Priority=1  SimulationMode=Phasor  SolverType=Tustin/Backward Euler (TBE)  SampleTime=50e-6  frequency=50  SPID=off  DisableSnubberDevices=off  DisableRonSwitches=off  DisableVfSwitches=off  SwTol=0  DisplayEquations=off  Interpol=off  ExternalGateDelay=off  methode=off  Ts=10  FunctionMessages=off  echomessages=off  HookPort=off  EnableUseOfTLC=off  x0status=blocks  frequencyindice=50  Pbase=3000e6  ErrMax=0.0001  Iterations=50  UnitsV=V  UnitsW=W  buscounter=0  RestoreLinks=warning  ResistiveCurrentMeasurement=off  Frange=[0:2:500]  Ylog=off  Xlog=on  ShowGrid=off  save=off  variable=ZData  structure=0  ZoomFFT=off  StartTime=0.0  cycles=1  DisplayStyle=1  fundamental=60  FreqAxis=off  MaxFrequency=1000  frequencyindicesteady=1  RmsSteady=1  display=off
  connections:
  _CN_169733763_132000_CN_171416196_132000/LConn1 -- T_169733763__/LConn1 -- _CN_169733763_132000_CN_224243440_132000/LConn1 -- _CN_169733763_132000_CN_151306638_132000/LConn1 -- _CN_169733763_132000_CN_171528627_132000/LConn1
  _CN_169733763_132000_CN_171416196_132000/LConn2 -- T_169733763__/LConn2 -- _CN_169733763_132000_CN_224243440_132000/LConn2 -- _CN_169733763_132000_CN_151306638_132000/LConn2 -- _CN_169733763_132000_CN_171528627_132000/LConn2
  _CN_169733763_132000_CN_171416196_132000/LConn3 -- T_169733763__/LConn3 -- _CN_169733763_132000_CN_224243440_132000/LConn3 -- _CN_169733763_132000_CN_151306638_132000/LConn3 -- _CN_169733763_132000_CN_171528627_132000/LConn3 -- bus1/LConn1
  _CN_169733763_132000_CN_171416196_132000/RConn1 -- T_171416196__/RConn1 -- _CN_171416196_132000_CN_171417653_132000/LConn1 -- L_171416196/LConn1
  _CN_169733763_132000_CN_171416196_132000/RConn2 -- T_171416196__/RConn2 -- _CN_171416196_132000_CN_171417653_132000/LConn2 -- L_171416196/LConn2
  _CN_169733763_132000_CN_171416196_132000/RConn3 -- T_171416196__/RConn3 -- _CN_171416196_132000_CN_171417653_132000/LConn3 -- L_171416196/LConn3 -- bus2/LConn1
  T_224243440__/LConn1 -- _CN_169733763_132000_CN_224243440_132000/RConn1
  T_224243440__/LConn2 -- _CN_169733763_132000_CN_224243440_132000/RConn2
  _CN_169733763_132000_CN_224243440_132000/RConn3 -- T_224243440__/LConn3 -- bus3/LConn1
  _CN_169733763_132000_CN_151306638_132000/RConn1 -- T_151306638__/LConn1 -- _CN_151306638_132000_CN_171367521_132000/LConn1
  _CN_169733763_132000_CN_151306638_132000/RConn2 -- T_151306638__/LConn2 -- _CN_151306638_132000_CN_171367521_132000/LConn2
  _CN_169733763_132000_CN_151306638_132000/RConn3 -- T_151306638__/LConn3 -- _CN_151306638_132000_CN_171367521_132000/LConn3 -- bus4/LConn1
  _CN_169733763_132000_CN_171528627_132000/RConn1 -- T_171528627__/LConn1 -- _CN_171528627_132000_CN_169725350_132000/LConn1
  _CN_169733763_132000_CN_171528627_132000/RConn2 -- T_171528627__/LConn2 -- _CN_171528627_132000_CN_169725350_132000/LConn2
  _CN_169733763_132000_CN_171528627_132000/RConn3 -- T_171528627__/LConn3 -- _CN_171528627_132000_CN_169725350_132000/LConn3 -- bus5/LConn1
  T_171417653__/LConn1 -- _CN_171416196_132000_CN_171417653_132000/RConn1
  T_171417653__/LConn2 -- _CN_171416196_132000_CN_171417653_132000/RConn2
  _CN_171416196_132000_CN_171417653_132000/RConn3 -- T_171417653__/LConn3 -- bus6/LConn1
  _CN_171528627_132000_CN_169725350_132000/RConn1 -- T_169725350__/LConn1 -- _CN_169725350_132000_CN_169848807_132000/LConn1
  _CN_171528627_132000_CN_169725350_132000/RConn2 -- T_169725350__/LConn2 -- _CN_169725350_132000_CN_169848807_132000/LConn2
  _CN_171528627_132000_CN_169725350_132000/RConn3 -- T_169725350__/LConn3 -- _CN_169725350_132000_CN_169848807_132000/LConn3 -- bus7/LConn1
  T_171367521__/LConn1 -- _CN_151306638_132000_CN_171367521_132000/RConn1
  T_171367521__/LConn2 -- _CN_151306638_132000_CN_171367521_132000/RConn2
  _CN_151306638_132000_CN_171367521_132000/RConn3 -- T_171367521__/LConn3 -- bus8/LConn1
  _CN_172334367_132000_CN_172341413_132000/LConn1 -- T_172334367__/LConn1 -- _CN_172334367_132000_CN_172539510_132000/LConn1
  _CN_172334367_132000_CN_172341413_132000/LConn2 -- T_172334367__/LConn2 -- _CN_172334367_132000_CN_172539510_132000/LConn2
  _CN_172334367_132000_CN_172341413_132000/LConn3 -- T_172334367__/LConn3 -- _CN_172334367_132000_CN_172539510_132000/LConn3 -- bus9/LConn1
  _CN_172334367_132000_CN_172341413_132000/RConn1 -- G_172341413_/RConn1 -- _CN_177038810_220000_CN_172341413_132000/LConn1 -- _CN_177038725_220000_CN_172341413_132000/LConn1 -- _CN_172341412_132000_CN_172341413_132000/LConn1 -- _CN_223146054_132000_CN_172341413_132000/LConn1
  _CN_172334367_132000_CN_172341413_132000/RConn2 -- G_172341413_/RConn2 -- _CN_177038810_220000_CN_172341413_132000/LConn2 -- _CN_177038725_220000_CN_172341413_132000/LConn2 -- _CN_172341412_132000_CN_172341413_132000/LConn2 -- _CN_223146054_132000_CN_172341413_132000/LConn2
  _CN_172334367_132000_CN_172341413_132000/RConn3 -- G_172341413_/RConn3 -- _CN_177038810_220000_CN_172341413_132000/LConn3 -- bus10/LConn1 -- _CN_177038725_220000_CN_172341413_132000/LConn3 -- _CN_172341412_132000_CN_172341413_132000/LConn3 -- _CN_223146054_132000_CN_172341413_132000/LConn3
  _CN_172334367_132000_CN_172539510_132000/RConn1 -- T_172539510__/LConn1 -- _CN_172539510_132000_CN_172295139_132000/LConn1
  _CN_172334367_132000_CN_172539510_132000/RConn2 -- T_172539510__/LConn2 -- _CN_172539510_132000_CN_172295139_132000/LConn2
  _CN_172334367_132000_CN_172539510_132000/RConn3 -- T_172539510__/LConn3 -- _CN_172539510_132000_CN_172295139_132000/LConn3 -- bus11/LConn1
  _CN_172341412_132000_CN_172341413_132000/RConn1 -- T_172341412__/LConn1 -- _CN_172341412_132000_CN_172470451_132000/LConn1
  _CN_172341412_132000_CN_172341413_132000/RConn2 -- T_172341412__/LConn2 -- _CN_172341412_132000_CN_172470451_132000/LConn2
  _CN_172341412_132000_CN_172341413_132000/RConn3 -- T_172341412__/LConn3 -- _CN_172341412_132000_CN_172470451_132000/LConn3 -- bus12/LConn1
  _CN_172341412_132000_CN_172470451_132000/RConn1 -- T_172470451__/LConn1 -- _CN_172470451_132000_CN_172839368_132000/LConn1
  _CN_172341412_132000_CN_172470451_132000/RConn2 -- T_172470451__/LConn2 -- _CN_172470451_132000_CN_172839368_132000/LConn2
  _CN_172341412_132000_CN_172470451_132000/RConn3 -- T_172470451__/LConn3 -- _CN_172470451_132000_CN_172839368_132000/LConn3 -- bus13/LConn1
  _CN_169725350_132000_CN_169848807_132000/RConn1 -- T_169848807__/LConn1 -- _CN_169722202_132000_CN_169848807_132000/LConn1
  _CN_169725350_132000_CN_169848807_132000/RConn2 -- T_169848807__/LConn2 -- _CN_169722202_132000_CN_169848807_132000/LConn2
  _CN_169725350_132000_CN_169848807_132000/RConn3 -- T_169848807__/LConn3 -- _CN_169722202_132000_CN_169848807_132000/LConn3 -- bus14/LConn1
  T_194416935__/LConn1 -- _CN_194416935_132000_CN_172295139_132000/LConn1
  T_194416935__/LConn2 -- _CN_194416935_132000_CN_172295139_132000/LConn2
  _CN_194416935_132000_CN_172295139_132000/LConn3 -- T_194416935__/LConn3 -- bus15/LConn1
  _CN_194416935_132000_CN_172295139_132000/RConn1 -- G_172295139_/RConn1 -- _CN_172539510_132000_CN_172295139_132000/RConn1 -- _CN_172578742_220000_CN_172295139_132000/LConn1 -- _CN_177038810_220000_CN_172295139_132000/LConn1 -- _CN_194381791_220000_CN_172295139_132000/LConn1
  _CN_194416935_132000_CN_172295139_132000/RConn2 -- G_172295139_/RConn2 -- _CN_172539510_132000_CN_172295139_132000/RConn2 -- _CN_172578742_220000_CN_172295139_132000/LConn2 -- _CN_177038810_220000_CN_172295139_132000/LConn2 -- _CN_194381791_220000_CN_172295139_132000/LConn2
  _CN_194416935_132000_CN_172295139_132000/RConn3 -- G_172295139_/RConn3 -- _CN_172539510_132000_CN_172295139_132000/RConn3 -- _CN_172578742_220000_CN_172295139_132000/LConn3 -- _CN_177038810_220000_CN_172295139_132000/LConn3 -- _CN_194381791_220000_CN_172295139_132000/LConn3 -- bus16/LConn1
  T_172839368__/LConn1 -- _CN_172470451_132000_CN_172839368_132000/RConn1
  T_172839368__/LConn2 -- _CN_172470451_132000_CN_172839368_132000/RConn2
  _CN_172470451_132000_CN_172839368_132000/RConn3 -- T_172839368__/LConn3 -- bus17/LConn1
  T_177038903__/LConn1 -- _CN_177038903_132000_CN_177109317_132000/LConn1
  T_177038903__/LConn2 -- _CN_177038903_132000_CN_177109317_132000/LConn2
  _CN_177038903_132000_CN_177109317_132000/LConn3 -- T_177038903__/LConn3 -- bus18/LConn1
  T_177109317__/LConn1 -- _CN_177038903_132000_CN_177109317_132000/RConn1
  T_177109317__/LConn2 -- _CN_177038903_132000_CN_177109317_132000/RConn2
  _CN_177038903_132000_CN_177109317_132000/RConn3 -- T_177109317__/LConn3 -- bus19/LConn1
  _CN_223146054_132000_CN_172341413_132000/RConn1 -- T_223146054__/LConn1 -- _CN_223146054_132000_CN_177209321_132000/LConn1
  _CN_223146054_132000_CN_172341413_132000/RConn2 -- T_223146054__/LConn2 -- _CN_223146054_132000_CN_177209321_132000/LConn2
  _CN_223146054_132000_CN_172341413_132000/RConn3 -- T_223146054__/LConn3 -- _CN_223146054_132000_CN_177209321_132000/LConn3 -- bus20/LConn1
  T_177209321__/LConn1 -- _CN_223146054_132000_CN_177209321_132000/RConn1
  T_177209321__/LConn2 -- _CN_223146054_132000_CN_177209321_132000/RConn2
  _CN_223146054_132000_CN_177209321_132000/RConn3 -- T_177209321__/LConn3 -- bus21/LConn1
  T_171541461__/LConn1 -- _CN_171541461_132000_CN_171536873_132000/LConn1
  T_171541461__/LConn2 -- _CN_171541461_132000_CN_171536873_132000/LConn2
  _CN_171541461_132000_CN_171536873_132000/LConn3 -- T_171541461__/LConn3 -- bus22/LConn1
  _CN_171541461_132000_CN_171536873_132000/RConn1 -- T_171536873__/LConn1 -- _CN_171536873_132000_CN_169848809_132000/LConn1
  _CN_171541461_132000_CN_171536873_132000/RConn2 -- T_171536873__/LConn2 -- _CN_171536873_132000_CN_169848809_132000/LConn2
  _CN_171541461_132000_CN_171536873_132000/RConn3 -- T_171536873__/LConn3 -- _CN_171536873_132000_CN_169848809_132000/LConn3 -- bus23/LConn1
  _CN_169722202_132000_CN_169848809_132000/LConn1 -- T_169722202__/LConn1 -- _CN_169722202_132000_CN_169848807_132000/RConn1
  _CN_169722202_132000_CN_169848809_132000/LConn2 -- T_169722202__/LConn2 -- _CN_169722202_132000_CN_169848807_132000/RConn2
  _CN_169722202_132000_CN_169848809_132000/LConn3 -- T_169722202__/LConn3 -- _CN_169722202_132000_CN_169848807_132000/RConn3 -- bus24/LConn1
  _CN_169722202_132000_CN_169848809_132000/RConn1 -- T_169848809__/LConn1 -- _CN_171536873_132000_CN_169848809_132000/RConn1
  _CN_169722202_132000_CN_169848809_132000/RConn2 -- T_169848809__/LConn2 -- _CN_171536873_132000_CN_169848809_132000/RConn2
  _CN_169722202_132000_CN_169848809_132000/RConn3 -- T_169848809__/LConn3 -- _CN_171536873_132000_CN_169848809_132000/RConn3 -- bus25/LConn1
  _CN_223679746_220000_CN_213917891_220000/LConn1 -- T_223679746__/RConn1 -- L_223679746/LConn1
  _CN_223679746_220000_CN_213917891_220000/LConn2 -- T_223679746__/RConn2 -- L_223679746/LConn2
  _CN_223679746_220000_CN_213917891_220000/LConn3 -- T_223679746__/RConn3 -- L_223679746/LConn3 -- bus26/LConn1
  _CN_223679746_220000_CN_213917891_220000/RConn1 -- T_213917891_220000_/LConn1 -- _CN_193503031_220000_CN_213917891_220000/LConn1 -- _CN_180468905_220000_CN_213917891_220000/LConn1
  _CN_223679746_220000_CN_213917891_220000/RConn2 -- T_213917891_220000_/LConn2 -- _CN_193503031_220000_CN_213917891_220000/LConn2 -- _CN_180468905_220000_CN_213917891_220000/LConn2
  _CN_223679746_220000_CN_213917891_220000/RConn3 -- T_213917891_220000_/LConn3 -- _CN_193503031_220000_CN_213917891_220000/LConn3 -- bus27/LConn1 -- _CN_180468905_220000_CN_213917891_220000/LConn3
  _CN_177038723_220000_CN_102272939_220000/LConn1 -- T_177038723_220000_/LConn1 -- _CN_177038723_220000_CN_102271992_220000/LConn1
  _CN_177038723_220000_CN_102272939_220000/LConn2 -- T_177038723_220000_/LConn2 -- _CN_177038723_220000_CN_102271992_220000/LConn2
  _CN_177038723_220000_CN_102272939_220000/LConn3 -- T_177038723_220000_/LConn3 -- _CN_177038723_220000_CN_102271992_220000/LConn3 -- bus28/LConn1
  _CN_177038723_220000_CN_102272939_220000/RConn1 -- T_102272939_220000_/LConn1 -- _CN_105024673_220000_CN_102272939_220000/LConn1 -- _CN_102272939_220000_CN_102271992_220000/LConn1
  _CN_177038723_220000_CN_102272939_220000/RConn2 -- T_102272939_220000_/LConn2 -- _CN_105024673_220000_CN_102272939_220000/LConn2 -- _CN_102272939_220000_CN_102271992_220000/LConn2
  _CN_177038723_220000_CN_102272939_220000/RConn3 -- T_102272939_220000_/LConn3 -- _CN_105024673_220000_CN_102272939_220000/LConn3 -- _CN_102272939_220000_CN_102271992_220000/LConn3 -- bus29/LConn1
  _CN_177038723_220000_CN_102271992_220000/RConn1 -- T_102271992_220000_/LConn1 -- _CN_172185378_220000_CN_102271992_220000/LConn1 -- _CN_102272939_220000_CN_102271992_220000/RConn1 -- _CN_177038800_220000_CN_102271992_220000/LConn1
  _CN_177038723_220000_CN_102271992_220000/RConn2 -- T_102271992_220000_/LConn2 -- _CN_172185378_220000_CN_102271992_220000/LConn2 -- _CN_102272939_220000_CN_102271992_220000/RConn2 -- _CN_177038800_220000_CN_102271992_220000/LConn2
  _CN_177038723_220000_CN_102271992_220000/RConn3 -- T_102271992_220000_/LConn3 -- _CN_172185378_220000_CN_102271992_220000/LConn3 -- _CN_102272939_220000_CN_102271992_220000/RConn3 -- _CN_177038800_220000_CN_102271992_220000/LConn3 -- bus30/LConn1
  _CN_171416196_220000_CN_169619943_220000/LConn1 -- T_171416196__/LConn1 -- _CN_171416196_220000_CN_151126418_220000/LConn1
  _CN_171416196_220000_CN_169619943_220000/LConn2 -- T_171416196__/LConn2 -- _CN_171416196_220000_CN_151126418_220000/LConn2
  _CN_171416196_220000_CN_169619943_220000/LConn3 -- T_171416196__/LConn3 -- _CN_171416196_220000_CN_151126418_220000/LConn3 -- bus31/LConn1
  _CN_171416196_220000_CN_169619943_220000/RConn1 -- T_169619943__/LConn1 -- _CN_151126418_220000_CN_169619943_220000/LConn1
  _CN_171416196_220000_CN_169619943_220000/RConn2 -- T_169619943__/LConn2 -- _CN_151126418_220000_CN_169619943_220000/LConn2
  _CN_171416196_220000_CN_169619943_220000/RConn3 -- T_169619943__/LConn3 -- _CN_151126418_220000_CN_169619943_220000/LConn3 -- bus32/LConn1
  _CN_171416196_220000_CN_151126418_220000/RConn1 -- T_151126418__/LConn1 -- _CN_151126418_220000_CN_169619943_220000/RConn1
  _CN_171416196_220000_CN_151126418_220000/RConn2 -- T_151126418__/LConn2 -- _CN_151126418_220000_CN_169619943_220000/RConn2
  _CN_171416196_220000_CN_151126418_220000/RConn3 -- T_151126418__/LConn3 -- _CN_151126418_220000_CN_169619943_220000/RConn3 -- bus33/LConn1
  T_177038725__/LConn1 -- _CN_177038725_220000_CN_172341413_132000/RConn1
  T_177038725__/LConn2 -- _CN_177038725_220000_CN_172341413_132000/RConn2
  _CN_177038725_220000_CN_172341413_132000/RConn3 -- T_177038725__/LConn3 -- bus34/LConn1
  _CN_128825607_220000_CN_108036550_220000/LConn1 -- T_128825607_220000_/LConn1 -- _CN_128825607_220000_CN_110677040_220000/LConn1
  _CN_128825607_220000_CN_108036550_220000/LConn2 -- T_128825607_220000_/LConn2 -- _CN_128825607_220000_CN_110677040_220000/LConn2
  _CN_128825607_220000_CN_108036550_220000/LConn3 -- T_128825607_220000_/LConn3 -- _CN_128825607_220000_CN_110677040_220000/LConn3 -- bus35/LConn1
  _CN_128825607_220000_CN_108036550_220000/RConn1 -- G_108036550_Tripoli_South_OCGT_Power_Plant_محطه_توليد_كهرباء_غازيه_جنوب_طرابلس/RConn1 -- _CN_106772180_220000_CN_108036550_220000/LConn1 -- _CN_214448787_220000_CN_108036550_220000/LConn1 -- _CN_107267089_220000_CN_108036550_220000/LConn1
  _CN_128825607_220000_CN_108036550_220000/RConn2 -- G_108036550_Tripoli_South_OCGT_Power_Plant_محطه_توليد_كهرباء_غازيه_جنوب_طرابلس/RConn2 -- _CN_106772180_220000_CN_108036550_220000/LConn2 -- _CN_214448787_220000_CN_108036550_220000/LConn2 -- _CN_107267089_220000_CN_108036550_220000/LConn2
  _CN_128825607_220000_CN_108036550_220000/RConn3 -- G_108036550_Tripoli_South_OCGT_Power_Plant_محطه_توليد_كهرباء_غازيه_جنوب_طرابلس/RConn3 -- _CN_106772180_220000_CN_108036550_220000/LConn3 -- bus36/LConn1 -- _CN_214448787_220000_CN_108036550_220000/LConn3 -- _CN_107267089_220000_CN_108036550_220000/LConn3
  _CN_128825607_220000_CN_110677040_220000/RConn1 -- T_110677040_220000_/LConn1 -- _CN_110677040_220000_CN_161963067_220000/LConn1
  _CN_128825607_220000_CN_110677040_220000/RConn2 -- T_110677040_220000_/LConn2 -- _CN_110677040_220000_CN_161963067_220000/LConn2
  _CN_128825607_220000_CN_110677040_220000/RConn3 -- T_110677040_220000_/LConn3 -- _CN_110677040_220000_CN_161963067_220000/LConn3 -- bus37/LConn1
  T_103998472_220000_/LConn1 -- _CN_103998472_220000_CN_173478530_220000/LConn1
  T_103998472_220000_/LConn2 -- _CN_103998472_220000_CN_173478530_220000/LConn2
  _CN_103998472_220000_CN_173478530_220000/LConn3 -- T_103998472_220000_/LConn3 -- bus38/LConn1
  _CN_103998472_220000_CN_173478530_220000/RConn1 -- G_173478530_/RConn1 -- _CN_177368453_220000_CN_173478530_220000/LConn1
  _CN_103998472_220000_CN_173478530_220000/RConn2 -- G_173478530_/RConn2 -- _CN_177368453_220000_CN_173478530_220000/LConn2
  _CN_103998472_220000_CN_173478530_220000/RConn3 -- G_173478530_/RConn3 -- _CN_177368453_220000_CN_173478530_220000/LConn3 -- bus39/LConn1
  _CN_217697930_220000_CN_213917888_220000/LConn1 -- T_217697930_220000_محطه_رفع_جهد_220/LConn1 -- _CN_217697930_220000_CN_193610426_220000/LConn1
  _CN_217697930_220000_CN_213917888_220000/LConn2 -- T_217697930_220000_محطه_رفع_جهد_220/LConn2 -- _CN_217697930_220000_CN_193610426_220000/LConn2
  _CN_217697930_220000_CN_213917888_220000/LConn3 -- T_217697930_220000_محطه_رفع_جهد_220/LConn3 -- _CN_217697930_220000_CN_193610426_220000/LConn3 -- bus40/LConn1
  _CN_217697930_220000_CN_213917888_220000/RConn1 -- G_213917888_/RConn1 -- _CN_193503031_220000_CN_213917888_220000/LConn1 -- _CN_193807037_220000_CN_213917888_220000/LConn1 -- _CN_364256186_220000_CN_213917888_220000/LConn1
  _CN_217697930_220000_CN_213917888_220000/RConn2 -- G_213917888_/RConn2 -- _CN_193503031_220000_CN_213917888_220000/LConn2 -- _CN_193807037_220000_CN_213917888_220000/LConn2 -- _CN_364256186_220000_CN_213917888_220000/LConn2
  _CN_217697930_220000_CN_213917888_220000/RConn3 -- G_213917888_/RConn3 -- _CN_193503031_220000_CN_213917888_220000/LConn3 -- _CN_193807037_220000_CN_213917888_220000/LConn3 -- _CN_364256186_220000_CN_213917888_220000/LConn3 -- bus41/LConn1
  T_193610426__/LConn1 -- _CN_217697930_220000_CN_193610426_220000/RConn1
  T_193610426__/LConn2 -- _CN_217697930_220000_CN_193610426_220000/RConn2
  _CN_217697930_220000_CN_193610426_220000/RConn3 -- T_193610426__/LConn3 -- bus42/LConn1
  T_180957591_220000_/LConn1 -- _CN_180957591_220000_CN_180843806_220000/LConn1
  T_180957591_220000_/LConn2 -- _CN_180957591_220000_CN_180843806_220000/LConn2
  _CN_180957591_220000_CN_180843806_220000/LConn3 -- T_180957591_220000_/LConn3 -- bus43/LConn1
  _CN_180957591_220000_CN_180843806_220000/RConn1 -- T_180843806_220000_/LConn1 -- _CN_180843806_220000_CN_181022450_220000/LConn1
  _CN_180957591_220000_CN_180843806_220000/RConn2 -- T_180843806_220000_/LConn2 -- _CN_180843806_220000_CN_181022450_220000/LConn2
  _CN_180957591_220000_CN_180843806_220000/RConn3 -- T_180843806_220000_/LConn3 -- _CN_180843806_220000_CN_181022450_220000/LConn3 -- bus44/LConn1
  _CN_107267089_220000_CN_108036550_220000/RConn1 -- T_107267089_220000_/LConn1 -- _CN_107267089_220000_CN_313517843_220000/LConn1
  _CN_107267089_220000_CN_108036550_220000/RConn2 -- T_107267089_220000_/LConn2 -- _CN_107267089_220000_CN_313517843_220000/LConn2
  _CN_107267089_220000_CN_108036550_220000/RConn3 -- T_107267089_220000_/LConn3 -- _CN_107267089_220000_CN_313517843_220000/LConn3 -- bus45/LConn1
  _CN_107267089_220000_CN_313517843_220000/RConn1 -- G_313517843_محطه_توليد_الكهرباء_غرب_طرابلس_tripoli_west_power_station/RConn1 -- _CN_152699771_220000_CN_313517843_220000/LConn1
  _CN_107267089_220000_CN_313517843_220000/RConn2 -- G_313517843_محطه_توليد_الكهرباء_غرب_طرابلس_tripoli_west_power_station/RConn2 -- _CN_152699771_220000_CN_313517843_220000/LConn2
  _CN_107267089_220000_CN_313517843_220000/RConn3 -- G_313517843_محطه_توليد_الكهرباء_غرب_طرابلس_tripoli_west_power_station/RConn3 -- _CN_152699771_220000_CN_313517843_220000/LConn3 -- bus46/LConn1
  _CN_214448787_220000_CN_152699771_220000/LConn1 -- T_214448787_220000_/LConn1 -- _CN_214448787_220000_CN_108036550_220000/RConn1
  _CN_214448787_220000_CN_152699771_220000/LConn2 -- T_214448787_220000_/LConn2 -- _CN_214448787_220000_CN_108036550_220000/RConn2
  _CN_214448787_220000_CN_152699771_220000/LConn3 -- T_214448787_220000_/LConn3 -- _CN_214448787_220000_CN_108036550_220000/RConn3 -- bus47/LConn1
  _CN_214448787_220000_CN_152699771_220000/RConn1 -- T_152699771__/LConn1 -- _CN_152699771_220000_CN_313517843_220000/RConn1
  _CN_214448787_220000_CN_152699771_220000/RConn2 -- T_152699771__/LConn2 -- _CN_152699771_220000_CN_313517843_220000/RConn2
  _CN_214448787_220000_CN_152699771_220000/RConn3 -- T_152699771__/LConn3 -- _CN_152699771_220000_CN_313517843_220000/RConn3 -- bus48/LConn1
  T_161956631__/LConn1 -- _CN_161956631_220000_CN_106772180_220000/LConn1
  T_161956631__/LConn2 -- _CN_161956631_220000_CN_106772180_220000/LConn2
  _CN_161956631_220000_CN_106772180_220000/LConn3 -- T_161956631__/LConn3 -- bus49/LConn1
  _CN_161956631_220000_CN_106772180_220000/RConn1 -- T_106772180__/LConn1 -- _CN_106772180_220000_CN_108036550_220000/RConn1 -- _CN_106772180_220000_CN_213839198_220000/LConn1 -- _CN_161963067_220000_CN_106772180_220000/LConn1
  _CN_161956631_220000_CN_106772180_220000/RConn2 -- T_106772180__/LConn2 -- _CN_106772180_220000_CN_108036550_220000/RConn2 -- _CN_106772180_220000_CN_213839198_220000/LConn2 -- _CN_161963067_220000_CN_106772180_220000/LConn2
  _CN_161956631_220000_CN_106772180_220000/RConn3 -- T_106772180__/LConn3 -- _CN_106772180_220000_CN_108036550_220000/RConn3 -- bus50/LConn1 -- _CN_106772180_220000_CN_213839198_220000/LConn3 -- _CN_161963067_220000_CN_106772180_220000/LConn3
  _CN_120090521_220000_CN_121506218_220000/LConn1 -- T_120090521__/LConn1 -- _CN_120090521_220000_CN_103283231_220000/LConn1
  _CN_120090521_220000_CN_121506218_220000/LConn2 -- T_120090521__/LConn2 -- _CN_120090521_220000_CN_103283231_220000/LConn2
  _CN_120090521_220000_CN_121506218_220000/LConn3 -- T_120090521__/LConn3 -- _CN_120090521_220000_CN_103283231_220000/LConn3 -- bus51/LConn1
  _CN_120090521_220000_CN_121506218_220000/RConn1 -- T_121506218_220000_/RConn1 -- _CN_121506218_220000_CN_213839198_220000/LConn1 -- _CN_121506218_220000_CN_181022450_220000/LConn1 -- L_121506218/LConn1 -- _CN_121506218_220000_CN_32961936_220000/LConn1
  _CN_120090521_220000_CN_121506218_220000/RConn2 -- T_121506218_220000_/RConn2 -- _CN_121506218_220000_CN_213839198_220000/LConn2 -- _CN_121506218_220000_CN_181022450_220000/LConn2 -- L_121506218/LConn2 -- _CN_121506218_220000_CN_32961936_220000/LConn2
  _CN_120090521_220000_CN_121506218_220000/RConn3 -- T_121506218_220000_/RConn3 -- _CN_121506218_220000_CN_213839198_220000/LConn3 -- _CN_121506218_220000_CN_181022450_220000/LConn3 -- L_121506218/LConn3 -- bus52/LConn1 -- _CN_121506218_220000_CN_32961936_220000/LConn3
  T_103283231__/LConn1 -- _CN_120090521_220000_CN_103283231_220000/RConn1
  T_103283231__/LConn2 -- _CN_120090521_220000_CN_103283231_220000/RConn2
  _CN_120090521_220000_CN_103283231_220000/RConn3 -- T_103283231__/LConn3 -- bus53/LConn1
  T_171952539__/LConn1 -- _CN_171952539_220000_CN_208406457_220000/LConn1
  T_171952539__/LConn2 -- _CN_171952539_220000_CN_208406457_220000/LConn2
  _CN_171952539_220000_CN_208406457_220000/LConn3 -- T_171952539__/LConn3 -- bus54/LConn1
  _CN_171952539_220000_CN_208406457_220000/RConn1 -- T_208406457__/LConn1 -- _CN_153222965_220000_CN_208406457_220000/LConn1
  _CN_171952539_220000_CN_208406457_220000/RConn2 -- T_208406457__/LConn2 -- _CN_153222965_220000_CN_208406457_220000/LConn2
  _CN_171952539_220000_CN_208406457_220000/RConn3 -- T_208406457__/LConn3 -- _CN_153222965_220000_CN_208406457_220000/LConn3 -- bus55/LConn1
  _CN_180843806_220000_CN_181022450_220000/RConn1 -- T_181022450_220000_/LConn1 -- _CN_194714166_220000_CN_181022450_220000/LConn1 -- _CN_121506218_220000_CN_181022450_220000/RConn1
  _CN_180843806_220000_CN_181022450_220000/RConn2 -- T_181022450_220000_/LConn2 -- _CN_194714166_220000_CN_181022450_220000/LConn2 -- _CN_121506218_220000_CN_181022450_220000/RConn2
  _CN_180843806_220000_CN_181022450_220000/RConn3 -- T_181022450_220000_/LConn3 -- _CN_194714166_220000_CN_181022450_220000/LConn3 -- bus56/LConn1 -- _CN_121506218_220000_CN_181022450_220000/RConn3
  T_105024673__/LConn1 -- _CN_105024673_220000_CN_102272939_220000/RConn1
  T_105024673__/LConn2 -- _CN_105024673_220000_CN_102272939_220000/RConn2
  _CN_105024673_220000_CN_102272939_220000/RConn3 -- T_105024673__/LConn3 -- bus57/LConn1
  _CN_172185378_220000_CN_102271992_220000/RConn1 -- T_172185378_220000_/LConn1 -- _CN_172185378_220000_CN_172085356_220000/LConn1
  _CN_172185378_220000_CN_102271992_220000/RConn2 -- T_172185378_220000_/LConn2 -- _CN_172185378_220000_CN_172085356_220000/LConn2
  _CN_172185378_220000_CN_102271992_220000/RConn3 -- T_172185378_220000_/LConn3 -- _CN_172185378_220000_CN_172085356_220000/LConn3 -- bus58/LConn1
  _CN_172185378_220000_CN_172085356_220000/RConn1 -- T_172085356_220000_/LConn1 -- _CN_177368453_220000_CN_172085356_220000/LConn1 -- _CN_218527311_220000_CN_172085356_220000/LConn1
  _CN_172185378_220000_CN_172085356_220000/RConn2 -- T_172085356_220000_/LConn2 -- _CN_177368453_220000_CN_172085356_220000/LConn2 -- _CN_218527311_220000_CN_172085356_220000/LConn2
  _CN_172185378_220000_CN_172085356_220000/RConn3 -- T_172085356_220000_/LConn3 -- _CN_177368453_220000_CN_172085356_220000/LConn3 -- _CN_218527311_220000_CN_172085356_220000/LConn3 -- bus59/LConn1
  T_214102064__/LConn1 -- _CN_214102064_220000_CN_218527311_220000/LConn1
  T_214102064__/LConn2 -- _CN_214102064_220000_CN_218527311_220000/LConn2
  _CN_214102064_220000_CN_218527311_220000/LConn3 -- T_214102064__/LConn3 -- bus60/LConn1
  _CN_214102064_220000_CN_218527311_220000/RConn1 -- T_218527311__/LConn1 -- _CN_218527311_220000_CN_172085356_220000/RConn1
  _CN_214102064_220000_CN_218527311_220000/RConn2 -- T_218527311__/LConn2 -- _CN_218527311_220000_CN_172085356_220000/RConn2
  _CN_214102064_220000_CN_218527311_220000/RConn3 -- T_218527311__/LConn3 -- _CN_218527311_220000_CN_172085356_220000/RConn3 -- bus61/LConn1
  _CN_180468905_220000_CN_181030546_220000/LConn1 -- T_180468905__/LConn1 -- _CN_180468905_220000_CN_180477877_220000/LConn1 -- _CN_180468905_220000_CN_213917891_220000/RConn1
  _CN_180468905_220000_CN_181030546_220000/LConn2 -- T_180468905__/LConn2 -- _CN_180468905_220000_CN_180477877_220000/LConn2 -- _CN_180468905_220000_CN_213917891_220000/RConn2
  _CN_180468905_220000_CN_181030546_220000/LConn3 -- T_180468905__/LConn3 -- _CN_180468905_220000_CN_180477877_220000/LConn3 -- _CN_180468905_220000_CN_213917891_220000/RConn3 -- bus62/LConn1
  _CN_180468905_220000_CN_181030546_220000/RConn1 -- T_181030546__/LConn1 -- _CN_172578742_220000_CN_181030546_220000/LConn1
  _CN_180468905_220000_CN_181030546_220000/RConn2 -- T_181030546__/LConn2 -- _CN_172578742_220000_CN_181030546_220000/LConn2
  _CN_180468905_220000_CN_181030546_220000/RConn3 -- T_181030546__/LConn3 -- _CN_172578742_220000_CN_181030546_220000/LConn3 -- bus63/LConn1
  T_180477877__/LConn1 -- _CN_180468905_220000_CN_180477877_220000/RConn1
  T_180477877__/LConn2 -- _CN_180468905_220000_CN_180477877_220000/RConn2
  _CN_180468905_220000_CN_180477877_220000/RConn3 -- T_180477877__/LConn3 -- bus64/LConn1
  G_32961936_Khoms_Power_Plant/RConn1 -- _CN_121506218_220000_CN_32961936_220000/RConn1
  G_32961936_Khoms_Power_Plant/RConn2 -- _CN_121506218_220000_CN_32961936_220000/RConn2
  _CN_121506218_220000_CN_32961936_220000/RConn3 -- G_32961936_Khoms_Power_Plant/RConn3 -- bus65/LConn1
  _CN_121506218_220000_CN_213839198_220000/RConn1 -- T_213839198_220000_/LConn1 -- _CN_106772180_220000_CN_213839198_220000/RConn1
  _CN_121506218_220000_CN_213839198_220000/RConn2 -- T_213839198_220000_/LConn2 -- _CN_106772180_220000_CN_213839198_220000/RConn2
  _CN_121506218_220000_CN_213839198_220000/RConn3 -- T_213839198_220000_/LConn3 -- _CN_106772180_220000_CN_213839198_220000/RConn3 -- bus66/LConn1
  _CN_110677040_220000_CN_161963067_220000/RConn1 -- T_161963067__/LConn1 -- _CN_161963067_220000_CN_106772180_220000/RConn1
  _CN_110677040_220000_CN_161963067_220000/RConn2 -- T_161963067__/LConn2 -- _CN_161963067_220000_CN_106772180_220000/RConn2
  _CN_110677040_220000_CN_161963067_220000/RConn3 -- T_161963067__/LConn3 -- _CN_161963067_220000_CN_106772180_220000/RConn3 -- bus67/LConn1
  T_169756849__/LConn1 -- _CN_169756849_220000_CN_194381791_220000/LConn1
  T_169756849__/LConn2 -- _CN_169756849_220000_CN_194381791_220000/LConn2
  _CN_169756849_220000_CN_194381791_220000/LConn3 -- T_169756849__/LConn3 -- bus68/LConn1
  _CN_169756849_220000_CN_194381791_220000/RConn1 -- T_194381791__/LConn1 -- _CN_194381791_220000_CN_172295139_132000/RConn1
  _CN_169756849_220000_CN_194381791_220000/RConn2 -- T_194381791__/LConn2 -- _CN_194381791_220000_CN_172295139_132000/RConn2
  _CN_169756849_220000_CN_194381791_220000/RConn3 -- T_194381791__/LConn3 -- _CN_194381791_220000_CN_172295139_132000/RConn3 -- bus69/LConn1
  _CN_153222965_220000_CN_208406457_220000/RConn1 -- T_153222965__/LConn1 -- _CN_153222965_220000_CN_161744923_220000/LConn1
  _CN_153222965_220000_CN_208406457_220000/RConn2 -- T_153222965__/LConn2 -- _CN_153222965_220000_CN_161744923_220000/LConn2
  _CN_153222965_220000_CN_208406457_220000/RConn3 -- T_153222965__/LConn3 -- _CN_153222965_220000_CN_161744923_220000/LConn3 -- bus70/LConn1
  G_161744923_/RConn1 -- _CN_153222965_220000_CN_161744923_220000/RConn1
  G_161744923_/RConn2 -- _CN_153222965_220000_CN_161744923_220000/RConn2
  _CN_153222965_220000_CN_161744923_220000/RConn3 -- G_161744923_/RConn3 -- bus71/LConn1
  _CN_172578742_220000_CN_181030546_220000/RConn1 -- T_172578742__/LConn1 -- _CN_172578742_220000_CN_172295139_132000/RConn1
  _CN_172578742_220000_CN_181030546_220000/RConn2 -- T_172578742__/LConn2 -- _CN_172578742_220000_CN_172295139_132000/RConn2
  _CN_172578742_220000_CN_181030546_220000/RConn3 -- T_172578742__/LConn3 -- _CN_172578742_220000_CN_172295139_132000/RConn3 -- bus72/LConn1
  _CN_193503031_220000_CN_213917891_220000/RConn1 -- T_193503031_220000_/LConn1 -- _CN_193503031_220000_CN_213917888_220000/RConn1
  _CN_193503031_220000_CN_213917891_220000/RConn2 -- T_193503031_220000_/LConn2 -- _CN_193503031_220000_CN_213917888_220000/RConn2
  _CN_193503031_220000_CN_213917891_220000/RConn3 -- T_193503031_220000_/LConn3 -- _CN_193503031_220000_CN_213917888_220000/RConn3 -- bus73/LConn1
  T_193807037__/LConn1 -- _CN_193807037_220000_CN_213917888_220000/RConn1
  T_193807037__/LConn2 -- _CN_193807037_220000_CN_213917888_220000/RConn2
  _CN_193807037_220000_CN_213917888_220000/RConn3 -- T_193807037__/LConn3 -- bus74/LConn1
  _CN_177368453_220000_CN_173478530_220000/RConn1 -- T_177368453_220000_/LConn1 -- _CN_177368453_220000_CN_172085356_220000/RConn1
  _CN_177368453_220000_CN_173478530_220000/RConn2 -- T_177368453_220000_/LConn2 -- _CN_177368453_220000_CN_172085356_220000/RConn2
  _CN_177368453_220000_CN_173478530_220000/RConn3 -- T_177368453_220000_/LConn3 -- _CN_177368453_220000_CN_172085356_220000/RConn3 -- bus75/LConn1
  T_194714166_220000_/LConn1 -- _CN_194714166_220000_CN_181022450_220000/RConn1
  T_194714166_220000_/LConn2 -- _CN_194714166_220000_CN_181022450_220000/RConn2
  _CN_194714166_220000_CN_181022450_220000/RConn3 -- T_194714166_220000_/LConn3 -- bus76/LConn1
  T_173952590__/LConn1 -- _CN_173952590_220000_CN_289415384_220000/LConn1
  T_173952590__/LConn2 -- _CN_173952590_220000_CN_289415384_220000/LConn2
  _CN_173952590_220000_CN_289415384_220000/LConn3 -- T_173952590__/LConn3 -- bus77/LConn1
  T_289415384__/LConn1 -- _CN_173952590_220000_CN_289415384_220000/RConn1
  T_289415384__/LConn2 -- _CN_173952590_220000_CN_289415384_220000/RConn2
  _CN_173952590_220000_CN_289415384_220000/RConn3 -- T_289415384__/LConn3 -- bus78/LConn1
  T_177038800__/LConn1 -- _CN_177038800_220000_CN_102271992_220000/RConn1
  T_177038800__/LConn2 -- _CN_177038800_220000_CN_102271992_220000/RConn2
  _CN_177038800_220000_CN_102271992_220000/RConn3 -- T_177038800__/LConn3 -- bus79/LConn1
  _CN_177038810_220000_CN_172341413_132000/RConn1 -- T_177038810__/RConn1 -- _CN_177038810_220000_CN_172295139_132000/RConn1 -- L_177038810/LConn1
  _CN_177038810_220000_CN_172341413_132000/RConn2 -- T_177038810__/RConn2 -- _CN_177038810_220000_CN_172295139_132000/RConn2 -- L_177038810/LConn2
  _CN_177038810_220000_CN_172341413_132000/RConn3 -- T_177038810__/RConn3 -- _CN_177038810_220000_CN_172295139_132000/RConn3 -- L_177038810/LConn3 -- bus80/LConn1
  T_364256186__/LConn1 -- _CN_364256186_220000_CN_213917888_220000/RConn1
  T_364256186__/LConn2 -- _CN_364256186_220000_CN_213917888_220000/RConn2
  _CN_364256186_220000_CN_213917888_220000/RConn3 -- T_364256186__/LConn3 -- bus81/LConn1
  T_171540563__/LConn1 -- _CN_171540563_400000_CN_171416195_400000/LConn1
  T_171540563__/LConn2 -- _CN_171540563_400000_CN_171416195_400000/LConn2
  _CN_171540563_400000_CN_171416195_400000/LConn3 -- T_171540563__/LConn3 -- bus82/LConn1
  T_171416195__/LConn1 -- _CN_171540563_400000_CN_171416195_400000/RConn1
  T_171416195__/LConn2 -- _CN_171540563_400000_CN_171416195_400000/RConn2
  _CN_171540563_400000_CN_171416195_400000/RConn3 -- T_171416195__/LConn3 -- bus83/LConn1
  _CN_213914980_400000_CN_121506218_400000/LConn1 -- T_213914980__/LConn1 -- _CN_213914980_400000_CN_223679746_400000/LConn1
  _CN_213914980_400000_CN_121506218_400000/LConn2 -- T_213914980__/LConn2 -- _CN_213914980_400000_CN_223679746_400000/LConn2
  _CN_213914980_400000_CN_121506218_400000/LConn3 -- T_213914980__/LConn3 -- _CN_213914980_400000_CN_223679746_400000/LConn3 -- bus84/LConn1
  _CN_213914980_400000_CN_121506218_400000/RConn1 -- T_121506218_220000_/LConn1 -- _CN_121506218_400000_CN_177539635_400000/LConn1
  _CN_213914980_400000_CN_121506218_400000/RConn2 -- T_121506218_220000_/LConn2 -- _CN_121506218_400000_CN_177539635_400000/LConn2
  _CN_213914980_400000_CN_121506218_400000/RConn3 -- T_121506218_220000_/LConn3 -- _CN_121506218_400000_CN_177539635_400000/LConn3 -- bus85/LConn1
  T_223679746__/LConn1 -- _CN_213914980_400000_CN_223679746_400000/RConn1
  T_223679746__/LConn2 -- _CN_213914980_400000_CN_223679746_400000/RConn2
  _CN_213914980_400000_CN_223679746_400000/RConn3 -- T_223679746__/LConn3 -- bus86/LConn1
  _CN_121506218_400000_CN_177539635_400000/RConn1 -- T_177539635__/LConn1 -- _CN_177539635_400000_CN_177038810_400000/LConn1
  _CN_121506218_400000_CN_177539635_400000/RConn2 -- T_177539635__/LConn2 -- _CN_177539635_400000_CN_177038810_400000/LConn2
  _CN_121506218_400000_CN_177539635_400000/RConn3 -- T_177539635__/LConn3 -- _CN_177539635_400000_CN_177038810_400000/LConn3 -- bus87/LConn1
  T_177038810__/LConn1 -- _CN_177539635_400000_CN_177038810_400000/RConn1
  T_177038810__/LConn2 -- _CN_177539635_400000_CN_177038810_400000/RConn2
  _CN_177539635_400000_CN_177038810_400000/RConn3 -- T_177038810__/LConn3 -- bus88/LConn1
  T_169733763__/RConn1 -- L_169733763/LConn1
  T_169733763__/RConn2 -- L_169733763/LConn2
  L_169733763/LConn3 -- T_169733763__/RConn3 -- bus89/LConn1
  T_224243440__/RConn1 -- L_224243440/LConn1
  T_224243440__/RConn2 -- L_224243440/LConn2
  L_224243440/LConn3 -- T_224243440__/RConn3 -- bus90/LConn1
  T_151306638__/RConn1 -- L_151306638/LConn1
  T_151306638__/RConn2 -- L_151306638/LConn2
  L_151306638/LConn3 -- T_151306638__/RConn3 -- bus91/LConn1
  T_171528627__/RConn1 -- L_171528627/LConn1
  T_171528627__/RConn2 -- L_171528627/LConn2
  L_171528627/LConn3 -- T_171528627__/RConn3 -- bus92/LConn1
  T_171417653__/RConn1 -- L_171417653/LConn1
  T_171417653__/RConn2 -- L_171417653/LConn2
  L_171417653/LConn3 -- T_171417653__/RConn3 -- bus93/LConn1
  T_169725350__/RConn1 -- L_169725350/LConn1
  T_169725350__/RConn2 -- L_169725350/LConn2
  L_169725350/LConn3 -- T_169725350__/RConn3 -- bus94/LConn1
  T_171367521__/RConn1 -- L_171367521/LConn1
  T_171367521__/RConn2 -- L_171367521/LConn2
  L_171367521/LConn3 -- T_171367521__/RConn3 -- bus95/LConn1
  T_172334367__/RConn1 -- L_172334367/LConn1
  T_172334367__/RConn2 -- L_172334367/LConn2
  L_172334367/LConn3 -- T_172334367__/RConn3 -- bus96/LConn1
  T_172539510__/RConn1 -- L_172539510/LConn1
  T_172539510__/RConn2 -- L_172539510/LConn2
  L_172539510/LConn3 -- T_172539510__/RConn3 -- bus97/LConn1
  T_172341412__/RConn1 -- L_172341412/LConn1
  T_172341412__/RConn2 -- L_172341412/LConn2
  L_172341412/LConn3 -- T_172341412__/RConn3 -- bus98/LConn1
  T_172470451__/RConn1 -- L_172470451/LConn1
  T_172470451__/RConn2 -- L_172470451/LConn2
  L_172470451/LConn3 -- T_172470451__/RConn3 -- bus99/LConn1
  T_169848807__/RConn1 -- L_169848807/LConn1
  T_169848807__/RConn2 -- L_169848807/LConn2
  L_169848807/LConn3 -- T_169848807__/RConn3 -- bus100/LConn1
  T_194416935__/RConn1 -- L_194416935/LConn1
  T_194416935__/RConn2 -- L_194416935/LConn2
  L_194416935/LConn3 -- T_194416935__/RConn3 -- bus101/LConn1
  T_172839368__/RConn1 -- L_172839368/LConn1
  T_172839368__/RConn2 -- L_172839368/LConn2
  L_172839368/LConn3 -- T_172839368__/RConn3 -- bus102/LConn1
  T_177038903__/RConn1 -- L_177038903/LConn1
  T_177038903__/RConn2 -- L_177038903/LConn2
  L_177038903/LConn3 -- T_177038903__/RConn3 -- bus103/LConn1
  T_177109317__/RConn1 -- L_177109317/LConn1
  T_177109317__/RConn2 -- L_177109317/LConn2
  L_177109317/LConn3 -- T_177109317__/RConn3 -- bus104/LConn1
  T_223146054__/RConn1 -- L_223146054/LConn1
  T_223146054__/RConn2 -- L_223146054/LConn2
  L_223146054/LConn3 -- T_223146054__/RConn3 -- bus105/LConn1
  T_177209321__/RConn1 -- L_177209321/LConn1
  T_177209321__/RConn2 -- L_177209321/LConn2
  L_177209321/LConn3 -- T_177209321__/RConn3 -- bus106/LConn1
  T_171541461__/RConn1 -- L_171541461/LConn1
  T_171541461__/RConn2 -- L_171541461/LConn2
  L_171541461/LConn3 -- T_171541461__/RConn3 -- bus107/LConn1
  T_171536873__/RConn1 -- L_171536873/LConn1
  T_171536873__/RConn2 -- L_171536873/LConn2
  L_171536873/LConn3 -- T_171536873__/RConn3 -- bus108/LConn1
  T_169722202__/RConn1 -- L_169722202/LConn1
  T_169722202__/RConn2 -- L_169722202/LConn2
  L_169722202/LConn3 -- T_169722202__/RConn3 -- bus109/LConn1
  T_169848809__/RConn1 -- L_169848809/LConn1
  T_169848809__/RConn2 -- L_169848809/LConn2
  L_169848809/LConn3 -- T_169848809__/RConn3 -- bus110/LConn1
  T_213917891_220000_/RConn1 -- L_213917891/LConn1
  T_213917891_220000_/RConn2 -- L_213917891/LConn2
  L_213917891/LConn3 -- T_213917891_220000_/RConn3 -- bus111/LConn1
  T_177038723_220000_/RConn1 -- L_177038723/LConn1
  T_177038723_220000_/RConn2 -- L_177038723/LConn2
  L_177038723/LConn3 -- T_177038723_220000_/RConn3 -- bus112/LConn1
  T_102272939_220000_/RConn1 -- L_102272939/LConn1
  T_102272939_220000_/RConn2 -- L_102272939/LConn2
  L_102272939/LConn3 -- T_102272939_220000_/RConn3 -- bus113/LConn1
  T_102271992_220000_/RConn1 -- L_102271992/LConn1
  T_102271992_220000_/RConn2 -- L_102271992/LConn2
  L_102271992/LConn3 -- T_102271992_220000_/RConn3 -- bus114/LConn1
  T_169619943__/RConn1 -- L_169619943/LConn1
  T_169619943__/RConn2 -- L_169619943/LConn2
  L_169619943/LConn3 -- T_169619943__/RConn3 -- bus115/LConn1
  T_151126418__/RConn1 -- L_151126418/LConn1
  T_151126418__/RConn2 -- L_151126418/LConn2
  L_151126418/LConn3 -- T_151126418__/RConn3 -- bus116/LConn1
  T_177038725__/RConn1 -- L_177038725/LConn1
  T_177038725__/RConn2 -- L_177038725/LConn2
  L_177038725/LConn3 -- T_177038725__/RConn3 -- bus117/LConn1
  T_128825607_220000_/RConn1 -- L_128825607/LConn1
  T_128825607_220000_/RConn2 -- L_128825607/LConn2
  L_128825607/LConn3 -- T_128825607_220000_/RConn3 -- bus118/LConn1
  T_110677040_220000_/RConn1 -- L_110677040/LConn1
  T_110677040_220000_/RConn2 -- L_110677040/LConn2
  L_110677040/LConn3 -- T_110677040_220000_/RConn3 -- bus119/LConn1
  T_103998472_220000_/RConn1 -- L_103998472/LConn1
  T_103998472_220000_/RConn2 -- L_103998472/LConn2
  L_103998472/LConn3 -- T_103998472_220000_/RConn3 -- bus120/LConn1
  T_217697930_220000_محطه_رفع_جهد_220/RConn1 -- L_217697930/LConn1
  T_217697930_220000_محطه_رفع_جهد_220/RConn2 -- L_217697930/LConn2
  L_217697930/LConn3 -- T_217697930_220000_محطه_رفع_جهد_220/RConn3 -- bus121/LConn1
  T_193610426__/RConn1 -- L_193610426/LConn1
  T_193610426__/RConn2 -- L_193610426/LConn2
  L_193610426/LConn3 -- T_193610426__/RConn3 -- bus122/LConn1
  T_180957591_220000_/RConn1 -- L_180957591/LConn1
  T_180957591_220000_/RConn2 -- L_180957591/LConn2
  L_180957591/LConn3 -- T_180957591_220000_/RConn3 -- bus123/LConn1
  T_180843806_220000_/RConn1 -- L_180843806/LConn1
  T_180843806_220000_/RConn2 -- L_180843806/LConn2
  L_180843806/LConn3 -- T_180843806_220000_/RConn3 -- bus124/LConn1
  T_107267089_220000_/RConn1 -- L_107267089/LConn1
  T_107267089_220000_/RConn2 -- L_107267089/LConn2
  L_107267089/LConn3 -- T_107267089_220000_/RConn3 -- bus125/LConn1
  T_214448787_220000_/RConn1 -- L_214448787/LConn1
  T_214448787_220000_/RConn2 -- L_214448787/LConn2
  L_214448787/LConn3 -- T_214448787_220000_/RConn3 -- bus126/LConn1
  T_152699771__/RConn1 -- L_152699771/LConn1
  T_152699771__/RConn2 -- L_152699771/LConn2
  L_152699771/LConn3 -- T_152699771__/RConn3 -- bus127/LConn1
  T_161956631__/RConn1 -- L_161956631/LConn1
  T_161956631__/RConn2 -- L_161956631/LConn2
  L_161956631/LConn3 -- T_161956631__/RConn3 -- bus128/LConn1
  T_106772180__/RConn1 -- L_106772180/LConn1
  T_106772180__/RConn2 -- L_106772180/LConn2
  L_106772180/LConn3 -- T_106772180__/RConn3 -- bus129/LConn1
  T_120090521__/RConn1 -- L_120090521/LConn1
  T_120090521__/RConn2 -- L_120090521/LConn2
  L_120090521/LConn3 -- T_120090521__/RConn3 -- bus130/LConn1
  T_103283231__/RConn1 -- L_103283231/LConn1
  T_103283231__/RConn2 -- L_103283231/LConn2
  L_103283231/LConn3 -- T_103283231__/RConn3 -- bus131/LConn1
  T_171952539__/RConn1 -- L_171952539/LConn1
  T_171952539__/RConn2 -- L_171952539/LConn2
  L_171952539/LConn3 -- T_171952539__/RConn3 -- bus132/LConn1
  T_208406457__/RConn1 -- L_208406457/LConn1
  T_208406457__/RConn2 -- L_208406457/LConn2
  L_208406457/LConn3 -- T_208406457__/RConn3 -- bus133/LConn1
  T_181022450_220000_/RConn1 -- L_181022450/LConn1
  T_181022450_220000_/RConn2 -- L_181022450/LConn2
  L_181022450/LConn3 -- T_181022450_220000_/RConn3 -- bus134/LConn1
  T_105024673__/RConn1 -- L_105024673/LConn1
  T_105024673__/RConn2 -- L_105024673/LConn2
  L_105024673/LConn3 -- T_105024673__/RConn3 -- bus135/LConn1
  T_172185378_220000_/RConn1 -- L_172185378/LConn1
  T_172185378_220000_/RConn2 -- L_172185378/LConn2
  L_172185378/LConn3 -- T_172185378_220000_/RConn3 -- bus136/LConn1
  T_172085356_220000_/RConn1 -- L_172085356/LConn1
  T_172085356_220000_/RConn2 -- L_172085356/LConn2
  L_172085356/LConn3 -- T_172085356_220000_/RConn3 -- bus137/LConn1
  T_214102064__/RConn1 -- L_214102064/LConn1
  T_214102064__/RConn2 -- L_214102064/LConn2
  L_214102064/LConn3 -- T_214102064__/RConn3 -- bus138/LConn1
  T_218527311__/RConn1 -- L_218527311/LConn1
  T_218527311__/RConn2 -- L_218527311/LConn2
  L_218527311/LConn3 -- T_218527311__/RConn3 -- bus139/LConn1
  T_180468905__/RConn1 -- L_180468905/LConn1
  T_180468905__/RConn2 -- L_180468905/LConn2
  L_180468905/LConn3 -- T_180468905__/RConn3 -- bus140/LConn1
  T_181030546__/RConn1 -- L_181030546/LConn1
  T_181030546__/RConn2 -- L_181030546/LConn2
  L_181030546/LConn3 -- T_181030546__/RConn3 -- bus141/LConn1
  T_180477877__/RConn1 -- L_180477877/LConn1
  T_180477877__/RConn2 -- L_180477877/LConn2
  L_180477877/LConn3 -- T_180477877__/RConn3 -- bus142/LConn1
  T_213839198_220000_/RConn1 -- L_213839198/LConn1
  T_213839198_220000_/RConn2 -- L_213839198/LConn2
  L_213839198/LConn3 -- T_213839198_220000_/RConn3 -- bus143/LConn1
  T_161963067__/RConn1 -- L_161963067/LConn1
  T_161963067__/RConn2 -- L_161963067/LConn2
  L_161963067/LConn3 -- T_161963067__/RConn3 -- bus144/LConn1
  T_169756849__/RConn1 -- L_169756849/LConn1
  T_169756849__/RConn2 -- L_169756849/LConn2
  L_169756849/LConn3 -- T_169756849__/RConn3 -- bus145/LConn1
  T_194381791__/RConn1 -- L_194381791/LConn1
  T_194381791__/RConn2 -- L_194381791/LConn2
  L_194381791/LConn3 -- T_194381791__/RConn3 -- bus146/LConn1
  T_153222965__/RConn1 -- L_153222965/LConn1
  T_153222965__/RConn2 -- L_153222965/LConn2
  L_153222965/LConn3 -- T_153222965__/RConn3 -- bus147/LConn1
  T_172578742__/RConn1 -- L_172578742/LConn1
  T_172578742__/RConn2 -- L_172578742/LConn2
  L_172578742/LConn3 -- T_172578742__/RConn3 -- bus148/LConn1
  T_193503031_220000_/RConn1 -- L_193503031/LConn1
  T_193503031_220000_/RConn2 -- L_193503031/LConn2
  L_193503031/LConn3 -- T_193503031_220000_/RConn3 -- bus149/LConn1
  T_193807037__/RConn1 -- L_193807037/LConn1
  T_193807037__/RConn2 -- L_193807037/LConn2
  L_193807037/LConn3 -- T_193807037__/RConn3 -- bus150/LConn1
  T_177368453_220000_/RConn1 -- L_177368453/LConn1
  T_177368453_220000_/RConn2 -- L_177368453/LConn2
  L_177368453/LConn3 -- T_177368453_220000_/RConn3 -- bus151/LConn1
  T_194714166_220000_/RConn1 -- L_194714166/LConn1
  T_194714166_220000_/RConn2 -- L_194714166/LConn2
  L_194714166/LConn3 -- T_194714166_220000_/RConn3 -- bus152/LConn1
  T_173952590__/RConn1 -- L_173952590/LConn1
  T_173952590__/RConn2 -- L_173952590/LConn2
  L_173952590/LConn3 -- T_173952590__/RConn3 -- bus153/LConn1
  T_289415384__/RConn1 -- L_289415384/LConn1
  T_289415384__/RConn2 -- L_289415384/LConn2
  L_289415384/LConn3 -- T_289415384__/RConn3 -- bus154/LConn1
  T_177038800__/RConn1 -- L_177038800/LConn1
  T_177038800__/RConn2 -- L_177038800/LConn2
  L_177038800/LConn3 -- T_177038800__/RConn3 -- bus155/LConn1
  T_364256186__/RConn1 -- L_364256186/LConn1
  T_364256186__/RConn2 -- L_364256186/LConn2
  L_364256186/LConn3 -- T_364256186__/RConn3 -- bus156/LConn1
  T_171540563__/RConn1 -- L_171540563/LConn1
  T_171540563__/RConn2 -- L_171540563/LConn2
  L_171540563/LConn3 -- T_171540563__/RConn3 -- bus157/LConn1
  T_171416195__/RConn1 -- L_171416195/LConn1
  T_171416195__/RConn2 -- L_171416195/LConn2
  L_171416195/LConn3 -- T_171416195__/RConn3 -- bus158/LConn1
  T_213914980__/RConn1 -- L_213914980/LConn1
  T_213914980__/RConn2 -- L_213914980/LConn2
  L_213914980/LConn3 -- T_213914980__/RConn3 -- bus159/LConn1
  T_177539635__/RConn1 -- L_177539635/LConn1
  T_177539635__/RConn2 -- L_177539635/LConn2
  L_177539635/LConn3 -- T_177539635__/RConn3 -- bus160/LConn1
